simulink library "ddm"  (R2021b)
settings: Solver=VariableStepAuto  StartTime=0.0  StopTime=10.0  RelTol=1e-3
undefined symbols (not defined in the file or in its folder): ENUM_ADASACCSTA_ERROR, ENUM_ADASACCSTA_OFF, ENUM_ADASACCSTA_STANDBY, ENUM_ADASISASTA_OFF, ENUM_ALLOWMOV_ALLOWREADY, ENUM_APS, ENUM_BRKSTA_ERROR, ENUM_BRKSTA_OFF, ENUM_BRKSTA_ON, ENUM_BRKSW_INVALID, ENUM_BRKSW_OFF, ENUM_BRKSW_ON, ENUM_CHGPREACTERRSTA_OBCPRE, ENUM_DCDCFAULTSTA_ANYFAULTLV1, ENUM_DCDCFAULTSTA_ANYFAULTLV2, ENUM_DRIVETRAIN_AWD, ENUM_DRIVETRAIN_FWD, ENUM_DRIVETRAIN_RWD, ENUM_DRSEATSTA_INVALID, ENUM_EDUDRTSTA_NORMAL, ENUM_EPBSTA_APPLIED, ENUM_EPBSTA_RELEASED, ENUM_HVBATTREADYPRE_READY, ENUM_MCUWARN_LV0, ENUM_MCUWARN_LV1, ENUM_MCUWARN_LV2, ENUM_MCUWARN_LV3, ENUM_MCUWARN_NOERROR, ENUM_OBCFAULTSTA_ANYFAULT, ENUM_PAS_R2F2, ENUM_PDFAULT_BATTPDFAIL, ENUM_PDFAULT_DCDCDISABLE, ENUM_PDFAULT_MCUDISABLE, ENUM_PDFAULT_MCUDISCHRG, ENUM_POWERSTA_OFF, ENUM_POWERSTA_ON, ENUM_POWERSTA_READY, ENUM_POWERSTA_STANDBY, ENUM_PRESSINDI_LOW, ENUM_PUFAULT_BATTUPFAIL, ENUM_PUFAULT_DCDCENABLEFAIL, ENUM_PUFAULT_PRECHRGCHKFAIL, ENUM_PUFAULT_SAFETYCHKFAIL, ENUM_PUSTATE_COMPLETED, ENUM_PWRSTASW_OFF, ENUM_PWRSTASW_OFFA, ENUM_PWRSTASW_OFFCHVCHRG, ENUM_PWRSTASW_OFFCLVCHRG, ENUM_PWRSTASW_ON, ENUM_PWRSTASW_ONHVCHRG, ENUM_PWRSTASW_READY, ENUM_PWRSTASW_STANDBY, ENUM_RANGESTA_12IN, ENUM_SHIFTCOMMAND_D, ENUM_SHIFTCOMMAND_N, ENUM_SHIFTCOMMAND_P, ENUM_SHIFTCOMMAND_R, ENUM_VEHMALFUNLV_2ND, ENUM_VEHMALFUNLV_3RD, ENUM_VEHMALFUNLV_4TH ... (+835)
libraries: hcu_lib x750, $bdroot x12, simulink x5
(part 2 of 28)

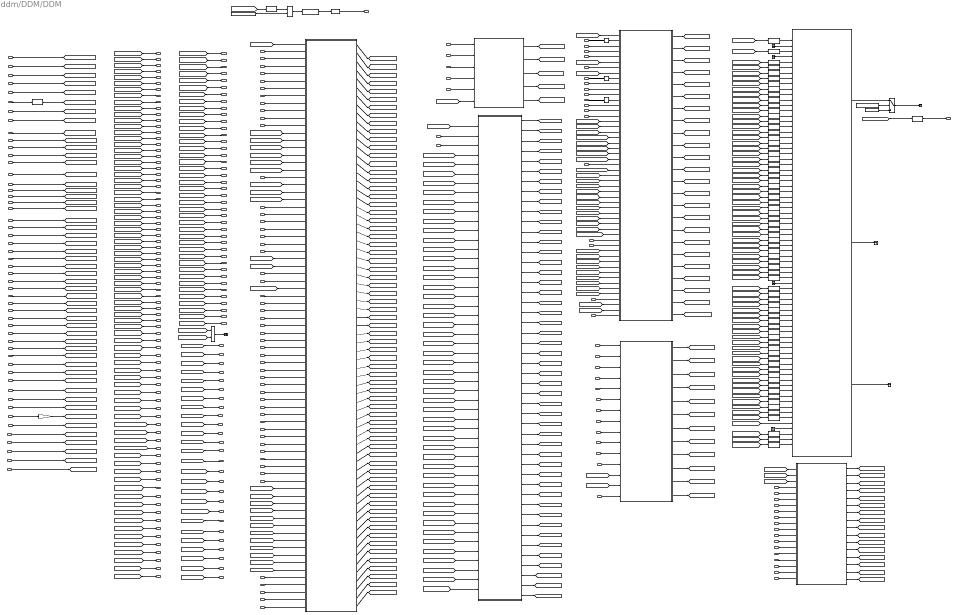
== system ddm/DDM/DDM ==
  task_time_s : Inport
  VINP_CANMsgValidABM1_flg : Inport  Port=2
  VINP_BrkPedalPosSta_enum : Inport  Port=3
  VINP_BrkPedalPos_pct : Inport  Port=4
  VINP_BrkSWSta_flg : Inport  Port=5
  VINP_CANMsgValidESC7_flg : Inport  Port=6
  VINP_CANMsgValidESC1_flg : Inport  Port=7
  VINP_CANMsgValidESC5_flg : Inport  Port=8
  VINP_CANMsgValidFCM2_flg : Inport  Port=9
  VINP_CANMsgValidFCM3_flg : Inport  Port=10
  VINP_CANMsgValidFCM4_flg : Inport  Port=11
  VINP_ADASACCSta_enum : Inport  Port=12
  VINP_VehSpeed_kph : Inport  Port=13
  VINP_ACCRequireAccel_mps2 : Inport  Port=14
  VDDM_ESC7RCErr_flg : Inport  Port=15
  VDDM_ESC7CSErr_flg : Inport  Port=16
  VDDM_ESC1RCErr_flg : Inport  Port=17
  VDDM_ESC1CSErr_flg : Inport  Port=18
  VDDM_ESC5RCErr_flg : Inport  Port=19
  VDDM_ESC5CSErr_flg : Inport  Port=20
  VDDM_FCM2RCErr_flg : Inport  Port=21
  VDDM_FCM2CSErr_flg : Inport  Port=22
  VDDM_FCM3RCErr_flg : Inport  Port=23
  VDDM_FCM3CSErr_flg : Inport  Port=24
  VDDM_FCM4CSErr_flg : Inport  Port=25
  VDDM_C1ABM1RCChk_flg : Inport  Port=26
  VDDM_C1ABM1CSChk_flg : Inport  Port=27
  VINP_CANMsgValidEPAS2_flg : Inport  Port=28
  VINP_EPBSta_enum : Inport  Port=29
  VDDM_FCM5CSErr_flg : Inport  Port=30
  VDDM_FCM5NoCom_flg : Inport  Port=31
  VINP_ADASISASta_enum : Inport  Port=32
  VINP_CANMsgValidBMS1_flg : Inport  Port=33
  VINP_CANMsgValidBMS6_flg : Inport  Port=34
  VINP_CANMsgValidCCU1_flg : Inport  Port=35
  VINP_CANMsgValidCCU2_flg : Inport  Port=36
  VINP_BMSWarn1_flg : Inport  Port=37
  VINP_BMSWarn2_flg : Inport  Port=38
  VINP_BMSWarn3_flg : Inport  Port=39
  VINP_BMSWarn4_flg : Inport  Port=40
  VINP_BMSWarn5_flg : Inport  Port=41
  VINP_BMSWarn6_flg : Inport  Port=42
  VINP_BMSWarn7_flg : Inport  Port=43
  VINP_BMSWarn8_flg : Inport  Port=44
  VINP_DCDCFaultSta_enum : Inport  Port=45
  VINP_OBCFaultSta_enum : Inport  Port=46
  VINP_MCUWarnF_enum : Inport  Port=47
  VINP_MCUWarnR_enum : Inport  Port=48
  VINP_LVBattDet12V_V : Inport  Port=49
  VINP_BMSREADY_flg : Inport  Port=50
  VINP_HVBattReady4Pre_enum : Inport  Port=51
  VINP_HVBContactorSta_flg : Inport  Port=52
  VINP_DCDCReady4Pre_flg : Inport  Port=53
  VINP_DCDCEnabled_flg : Inport  Port=54
  VINP_CANMsgValidBMS2_flg : Inport  Port=55
  VINP_CANMsgValidMCUF1_flg : Inport  Port=56
  VINP_CANMsgValidMCUR1_flg : Inport  Port=57
  VINP_CANMsgValidShifter1_flg : Inport  Port=58
  VINP_FrEDUDrtSta_flg : Inport  Port=59
  VINP_FrEDURealTMTq_Nm : Inport  Port=60
  VINP_RrEDUDrtSta_flg : Inport  Port=61
  VINP_RrEDURealTMTq_Nm : Inport  Port=62
  VDDM_C3BMS6RCChk_flg : Inport  Port=63
  VDDM_C3BMS6CSChk_flg : Inport  Port=64
  VDDM_C3BMS1RCChk_flg : Inport  Port=65
  VDDM_C3BMS1CSChk_flg : Inport  Port=66
  VDDM_C3CCU1RCChk_flg : Inport  Port=67
  VDDM_C3CCU1CSChk_flg : Inport  Port=68
  VDDM_C3CCU2RCChk_flg : Inport  Port=69
  VDDM_C3CCU2CSChk_flg : Inport  Port=70
  VDDM_MCUF1RCErr_flg : Inport  Port=71
  VDDM_MCUF1CSErr_flg : Inport  Port=72
  VDDM_MCUR1RCErr_flg : Inport  Port=73
  VDDM_MCUR1CSErr_flg : Inport  Port=74
  VDDM_Shifter1RCErr_flg : Inport  Port=75
  VDDM_Shifter1CSErr_flg : Inport  Port=76
  VINP_HVBattSOC_pct : Inport  Port=77
  VINP_ShifterHandleCmd_enum : Inport  Port=78
  VPMM_PowerSta_enum : Inport  Port=79
  VPMM_PwrStaSW_enum : Inport  Port=80
  VPMM_PowerUpFault_enum : Inport  Port=81
  VPMM_PowerDownFault_enum : Inport  Port=82
  VPMM_DrivetrainSelect_enum : Inport  Port=83
  VPMM_SafetyChkHLv_flg : Inport  Port=84
  VPMM_SafetyChkMLv_flg : Inport  Port=85
  VPMM_HVChrgPreActionErrSta_enum : Inport  Port=86
  VPMM_MCUReady_flg : Inport  Port=87
  VPMM_MCUReady4Pre_flg : Inport  Port=88
  VPMM_PowerUpState_enum : Inport  Port=89
  VPMM_MCUDCBusMaxVolt_V : Inport  Port=90
  VINP_BrakeSWGPIO_flg : Inport  Port=91
  VINP_BrakeLampSW_flg : Inport  Port=92
  VINP_DrStSW : Inport  Port=93
  VINP_FLAJARSW : Inport  Port=94
  VINP_FRAJARSW : Inport  Port=95
  VINP_RLAJARSW : Inport  Port=96
  VINP_RRAJARSW : Inport  Port=97
  VINP_HoodSW : Inport  Port=98
  VINP_TailgaSW : Inport  Port=99
  VINP_AccelPedal1Vol_V : Inport  Port=100
  VINP_AccelPedal2Vol_V : Inport  Port=101
  VDKC_DKCAuthSta_enum : Inport  Port=102
  VINP_AllowMovThd_OTA_enum : Inport  Port=103
  VINP_Pedal1Ref5V_V : Inport  Port=104
  VINP_Pedal2Ref5V_V : Inport  Port=105
  VINP_AuxBattVolmV_mV : Inport  Port=106
  No_CAN1_BUS_OFF : Inport  Port=107
  No_CAN3_BUS_OFF : Inport  Port=108
  No_CAN4_BUS_OFF : Inport  Port=109
  No_CAN_BUS_OFF : Inport  Port=110
  DTC_clear_request : Inport  Port=111
  VDHP_EAPCRBAD_flg : Inport  Port=112
  VDHP_EAPS12RangeSta_enum : Inport  Port=113
  VBCM_DiagHCrash_flg : Inport  Port=114
  VBCM_DiagFLTS_flg : Inport  Port=115
  VBCM_DiagFRTS_flg : Inport  Port=116
  VBCM_DiagRLTS_flg : Inport  Port=117
  VBCM_DiagRRTS_flg : Inport  Port=118
  VAPM_USSStaFCL_flg : Inport  Port=119
  VAPM_USSStaFML_flg : Inport  Port=120
  VAPM_USSStaFMR_flg : Inport  Port=121
  VAPM_USSStaFCR_flg : Inport  Port=122
  VAPM_USSStaRCL_flg : Inport  Port=123
  VAPM_USSStaRML_flg : Inport  Port=124
  VAPM_USSStaRMR_flg : Inport  Port=125
  VAPM_USSStaRCR_flg : Inport  Port=126
  VAPM_USSStaFLL_flg : Inport  Port=127
  VAPM_USSStaFLR_flg : Inport  Port=128
  VAPM_USSStaRLL_flg : Inport  Port=129
  VAPM_USSStaRLR_flg : Inport  Port=130
  VAPM_SNSRLayout_enum : Inport  Port=131
  VINP_ZoneSpdCtrlMode_enum : Inport  Port=132
  VDDM_ZoneSCPNoCom_flg : Inport  Port=133
  VINP_DrStdAErrSta_enum : Inport  Port=134
  VINP_ZoneDrMalfunLevel_enum : Inport  Port=135
  VINP_CANMsgValidDKC1_flg : Inport  Port=136
  VINP_CANMsgValidDKC2_flg : Inport  Port=137
  VVMC_ADASActive_flg : Inport  Port=138
  VTQR_FrTMTqReq_Nm : Inport  Port=139
  VTQR_RrTMTqReq_Nm : Inport  Port=140
  VTPM_LFBatwarn_flg : Inport  Port=141
  VTPM_RFBatwarn_flg : Inport  Port=142
  VTPM_LRBatwarn_flg : Inport  Port=143
  VTPM_RRBatwarn_flg : Inport  Port=144
  VTPM_LFPressIndi_enum : Inport  Port=145
  VTPM_RFPressIndi_enum : Inport  Port=146
  VTPM_LRPressIndi_enum : Inport  Port=147
  VTPM_RRPressIndi_enum : Inport  Port=148
  VTPM_LFWheelTmpIndi_flg : Inport  Port=149
  VTPM_RFWheelTmpIndi_flg : Inport  Port=150
  VTPM_LRWheelTmpIndi_flg : Inport  Port=151
  VTPM_RRWheelTmpIndi_flg : Inport  Port=152
  VTPM_LFSensorFail_flg : Inport  Port=153
  VTPM_RFSensorFail_flg : Inport  Port=154
  VTPM_LRSensorFail_flg : Inport  Port=155
  VTPM_RRSensorFail_flg : Inport  Port=156
  VTQD_ActParkRequest_flg : Inport  Port=157
  APM : Subsystem
  BCM : Subsystem
  Chart : Stateflow chart  TreatAsAtomicUnit=on
      settings: PortSchema="{\"entries\":[{\"content\":{\"sides\":[{\"content\":{\"connectorIds\":[]},\"type\":\"ConnectorPlacement.EquallySpacedRectSide\",\"uuid\":\"5c49d68c-3a13-4722-ae51-60c531d65ae1\"},{\"content\":{\"connectorIds\":[],\"side\":\"RIGHT\"},\"type\":\"ConnectorPlacement.EquallySpacedRectSide\",\"uuid\":\"1499f12d-58db-4e43-953b-81e532540c9e\"},{\"content\":{\"connectorIds\":[\"Out1\",\"Out2\",\"Out3\"],\"side\":\"TOP\"},\"type\":\"ConnectorPlacement.EquallySpacedRectSide\",\"uuid\":\"b40fb5a5-59a6-496c-b268-75370edec7d4\"},{\"content\":{\"connectorIds\":[\"In2\",\"In3\",\"In4\",\"In5\",\"In6\",\"In7\",\"In8\",\"In9\",\"In10\",\"In11\",\"In12\",\"In13\",\"In14\",\"In15\",\"In16\",\"In17\",\"In18\",\"In19\",\"In20\",\"In21\",\"In22\",\"In23\",\"In24\",\"In25\",\"In26\",\"In27\",\"In28\",\"In29\",\"In30\",\"In31\",\"In32\",\"In33\",\"In34\",\"In35\",\"In36\",\"In37\",\"In38\",\"In39\",\"In40\",\"In41\",\"In42\",\"In43\",\"In44\",\"In45\",\"In46\",\"In47\",\"In48\",\"In49\",\"In50\",\"In51\",\"In52\",\"In1\",\"In53\",\"In54\",\"In55\",\"In56\",\"In57\",\"In58\",\"In59\",\"In60\",\"In61\",\"In62\",\"In63\",\"In64\",\"In65\",\"In66\",\"In67\",\"In68\",\"In69\",\"In70\",\"In71\",\"In72\",\"In73\",\"In74\",\"In75\",\"In76\"],\"side\":\"BOTTOM\"},\"type\":\"ConnectorPlacement.EquallySpacedRectSide\",\"uuid\":\"7a3e18bf-6f06-4df1-889c-341cd16aa4bd\"}]},\"type\":\"ConnectorPlacement.EquallySpacedConnector\",\"uuid\":\"c096d691-37a2-471f-9d84-793135a13589\"}],\"packageUris\":[\"http://schema.mathworks.com/mf0/Connector/R2020b\"],\"version\":\"1.0\"}"
  Constant : Constant  Value=ENUM_PWRSTASW_READY
  Constant1 : Constant  Value=ZERO_INT
  Constant15 : Constant  Value=KDDM_VehMalfunLevelSW_flg
  Data Type Conversion{,1..48,50..72} (72 alike) : DataTypeConversion  OutDataTypeStr=boolean
  Data Type Conversion49 : DataTypeConversion  OutDataTypeStr=uint8
  Data Type Conversion73 : DataTypeConversion  OutDataTypeStr=uint8
  Detect Increase : simulink/Logic and Bit Operations/Detect Increase  vinit=0.0  OutDataTypeStr=boolean
  Equal : RelationalOperator  Operator===  OutDataTypeStr=boolean  RndMeth=Simplest
  Gain : Gain  Gain=XX2KXX
  Ground{1,3..4,26} (4 alike) : Ground
  Latch : hcu_lib/Basic_Blocks/Latch
  Logical Operator : Logic  Operator=NOT  AllPortsSameDT=off  OutDataTypeStr=boolean
  Logical Operator1 : Logic  Operator=NOT  AllPortsSameDT=off  OutDataTypeStr=boolean
  Logical Operator2 : Logic  Operator=NOT  AllPortsSameDT=off  OutDataTypeStr=boolean
  Logical Operator5 : Logic  Operator=OR  AllPortsSameDT=off  OutDataTypeStr=boolean
  PMM : Subsystem
  Switch : Switch  Criteria=u2 > Threshold
  TPM : Subsystem
  TQD : Subsystem
  Terminator{,1..3} (4 alike) : Terminator
  VMC_DDM : Subsystem
  VDDM_C3BMS6RCDTC_raw32 : Outport
  VDDM_C3BMS6CSDTC_raw32 : Outport  Port=2
  VDDM_C3BMS6LCDTC_raw32 : Outport  Port=3
  VDDM_C3BMS1RCDTC_raw32 : Outport  Port=4
  VDDM_C3BMS1CSDTC_raw32 : Outport  Port=5
  VDDM_C3BMS1LCDTC_raw32 : Outport  Port=6
  VDDM_C3CCU1RCDTC_raw32 : Outport  Port=7
  VDDM_C3CCU1CSDTC_raw32 : Outport  Port=8
  VDDM_C3CCU1LCDTC_raw32 : Outport  Port=9
  VDDM_C3CCU2RCDTC_raw32 : Outport  Port=10
  VDDM_C3CCU2CSDTC_raw32 : Outport  Port=11
  VDDM_C3CCU2LCDTC_raw32 : Outport  Port=12
  VDDM_C1ABM1RCDTC_raw32 : Outport  Port=13
  VDDM_C1ABM1CSDTC_raw32 : Outport  Port=14
  VDDM_C1ABM1LCDTC_raw32 : Outport  Port=15
  VDDM_Lv1ErrDTC_raw32 : Outport  Port=16
  VDDM_Lv2ErrDTC_raw32 : Outport  Port=17
  VDDM_Lv3ErrDTC_raw32 : Outport  Port=18
  VDDM_Lv4ErrDTC_raw32 : Outport  Port=19
  VDDM_BrkSWErrDTC_raw32 : Outport  Port=20
  VDDM_BrkSWNoBacDTC_raw32 : Outport  Port=21
  VDDM_KeyAuthDTC_raw32 : Outport  Port=22
  VDDM_ONtoRdyDTC_raw32 : Outport  Port=23
  VDDM_HVB4PreDTC_raw32 : Outport  Port=24
  VDDM_MCU4PreDTC_raw32 : Outport  Port=25
  VDDM_DCDC4PreDTC_raw32 : Outport  Port=26
  VDDM_HVRlyCloDTC_raw32 : Outport  Port=27
  VDDM_BMSRdyDTC_raw32 : Outport  Port=28
  VDDM_DCDCEnaDTC_raw32 : Outport  Port=29
  VDDM_HiLvSaChkDTC_raw32 : Outport  Port=30
  VDDM_MidLvSaChkDTC_raw32 : Outport  Port=31
  VDDM_MCUDisDTC_raw32 : Outport  Port=32
  VDDM_DCDCDisDTC_raw32 : Outport  Port=33
  VDDM_HVRlyOpDTC_raw32 : Outport  Port=34
  VDDM_MCUActDTC_raw32 : Outport  Port=35
  VDDM_OBC4PreDTC_raw32 : Outport  Port=36
  VDDM_IniLVLoDTC_raw32 : Outport  Port=37
  VDDM_LVSupLoDTC_raw32 : Outport  Port=38
  VDDM_LVSupHiDTC_raw32 : Outport  Port=39
  VDDM_DrStSWDTC_raw32 : Outport  Port=40
  VDDM_FLDoorSWDTC_raw32 : Outport  Port=41
  VDDM_RLDoorSWDTC_raw32 : Outport  Port=42
  VDDM_FRDoorSWDTC_raw32 : Outport  Port=43
  VDDM_RRDoorSWDTC_raw32 : Outport  Port=44
  VDDM_HoodSWDTC_raw32 : Outport  Port=45
  VDDM_TailgaSWDTC_raw32 : Outport  Port=46
  VDDM_VehMalfunLevel_enum : Outport  Port=47
  VDDM_APS1SigOoRDTC_raw32 : Outport  Port=48
  VDDM_APS2SigOoRDTC_raw32 : Outport  Port=49
  VDDM_APSCorrErrDTC_raw32 : Outport  Port=50
  VDDM_MCUF1NoComDTC_raw32 : Outport  Port=51
  VDDM_MCUR1NoComDTC_raw32 : Outport  Port=52
  VDDM_Shifter1NoComDTC_raw32 : Outport  Port=53
  VDDM_ESC7NoComDTC_raw32 : Outport  Port=54
  VDDM_ESC1NoComDTC_raw32 : Outport  Port=55
  VDDM_ESC5NoComDTC_raw32 : Outport  Port=56
  VDDM_EnterNewOperCyc_flg : Outport  Port=57
  VDDM_DiagHCrashDTC_raw32 : Outport  Port=58
  VDDM_DiagFLTSDTC_raw32 : Outport  Port=59
  VDDM_DiagFRTSDTC_raw32 : Outport  Port=60
  VDDM_DiagRLTSDTC_raw32 : Outport  Port=61
  VDDM_DiagRRTSDTC_raw32 : Outport  Port=62
  VDDM_FCLUSSDTC_raw32 : Outport  Port=63
  VDDM_FMLUSSDTC_raw32 : Outport  Port=64
  VDDM_FMRUSSDTC_raw32 : Outport  Port=65
  VDDM_FCRUSSDTC_raw32 : Outport  Port=66
  VDDM_RCLUSSDTC_raw32 : Outport  Port=67
  VDDM_RMLUSSDTC_raw32 : Outport  Port=68
  VDDM_RMRUSSDTC_raw32 : Outport  Port=69
  VDDM_RCRUSSDTC_raw32 : Outport  Port=70
  VDDM_FLLUSSDTC_raw32 : Outport  Port=71
  VDDM_FLRUSSDTC_raw32 : Outport  Port=72
  VDDM_RLLUSSDTC_raw32 : Outport  Port=73
  VDDM_RLRUSSDTC_raw32 : Outport  Port=74
  VDDM_FCM2NoComDTC_raw32 : Outport  Port=75
  VDDM_FCM2RCErrDTC_raw32 : Outport  Port=76
  VDDM_FCM2CSErrDTC_raw32 : Outport  Port=77
  VDDM_FCM3NoComDTC_raw32 : Outport  Port=78
  VDDM_FCM3RCErrDTC_raw32 : Outport  Port=79
  VDDM_FCM3CSErrDTC_raw32 : Outport  Port=80
  VDDM_FCM4NoComDTC_raw32 : Outport  Port=81
  VDDM_FCM4CSErrDTC_raw32 : Outport  Port=82
  VDDM_FCM5NoComDTC_raw32 : Outport  Port=83
  VDDM_FCM5CSErrDTC_raw32 : Outport  Port=84
  VDDM_ZoneSCPNoComDTC_raw32 : Outport  Port=85
  VDDM_BMSSigErrDetDTC_raw32 : Outport  Port=86
  VDDM_FCMACCSigErrDetDTC_raw32 : Outport  Port=87
  VDDM_FrMCUSigErrDetDTC_raw32 : Outport  Port=88
  VDDM_RrMCUSigErrDetDTC_raw32 : Outport  Port=89
  VDDM_CCUSigErrDetDTC_raw32 : Outport  Port=90
  VDDM_ACCAccelCmdErrDetDTC_raw32 : Outport  Port=91
  VDDM_ACCMalfuncDetDTC_raw32 : Outport  Port=92
  VDDM_CCMalfuncDetDTC_raw32 : Outport  Port=93
  VDDM_MSAMalfuncDetDTC_raw32 : Outport  Port=94
  VDDM_ISAMalfuncDetDTC_raw32 : Outport  Port=95
  VDDM_MCUF1RCErrDTC_raw32 : Outport  Port=96
  VDDM_MCUR1RCErrDTC_raw32 : Outport  Port=97
  VDDM_MCUF1CSErrDTC_raw32 : Outport  Port=98
  VDDM_MCUR1CSErrDTC_raw32 : Outport  Port=99
  VDDM_Shifter1RCErrDTC_raw32 : Outport  Port=100
  VDDM_Shifter1CSErrDTC_raw32 : Outport  Port=101
  VDDM_ESC7RCErrDTC_raw32 : Outport  Port=102
  VDDM_ESC7CSErrDTC_raw32 : Outport  Port=103
  VDDM_ESC1RCErrDTC_raw32 : Outport  Port=104
  VDDM_ESC1CSErrDTC_raw32 : Outport  Port=105
  VDDM_ESC5RCErrDTC_raw32 : Outport  Port=106
  VDDM_ESC5CSErrDTC_raw32 : Outport  Port=107
  VDDM_FrMCUTqErrDTC_raw32 : Outport  Port=108
  VDDM_RrMCUTqErrDTC_raw32 : Outport  Port=109
  VDDM_LFBatwarnDTC_raw32 : Outport  Port=110
  VDDM_RFBatwarnDTC_raw32 : Outport  Port=111
  VDDM_LRBatwarnDTC_raw32 : Outport  Port=112
  VDDM_RRBatwarnDTC_raw32 : Outport  Port=113
  VDDM_LFPressIndiDTC_raw32 : Outport  Port=114
  VDDM_RFPressIndiDTC_raw32 : Outport  Port=115
  VDDM_LRPressIndiDTC_raw32 : Outport  Port=116
  VDDM_RRPressIndiDTC_raw32 : Outport  Port=117
  VDDM_LFWheelTmpHighDTC_raw32 : Outport  Port=118
  VDDM_RFWheelTmpHighDTC_raw32 : Outport  Port=119
  VDDM_LRWheelTmpHighDTC_raw32 : Outport  Port=120
  VDDM_RRWheelTmpHighDTC_raw32 : Outport  Port=121
  VDDM_LFSensorFailDTC_raw32 : Outport  Port=122
  VDDM_RFSensorFailDTC_raw32 : Outport  Port=123
  VDDM_LRSensorFailDTC_raw32 : Outport  Port=124
  VDDM_RRSensorFailDTC_raw32 : Outport  Port=125
  VDDM_C1EPAS2LCDTC_raw32 : Outport  Port=126
  VDDM_5vAPS1PwrErrDTC_raw32 : Outport  Port=127
  VDDM_5vAPS2PwrErrDTC_raw32 : Outport  Port=128
  VDDM_EPBLockTODTC_raw32 : Outport  Port=129
  VDDM_EPBUnlockTODTC_raw32 : Outport  Port=130
  VDDM_HVRlyOpCFS_flg : Outport  Port=131
  VDDM_MCUActCFS_flg : Outport  Port=132
  VDDM_VCUACCErr_flg : Outport  Port=133
  VDDM_VCUISAErr_flg : Outport  Port=134
  VDDM_HVRlyOpFail_flg : Outport  Port=135
  VDDM_MCUActDisFail_flg : Outport  Port=136
  VDDM_VCUBrkSWSta_enum : Outport  Port=137
  VDDM_DrSeatSta_enum : Outport  Port=138
  VDDM_VCUFLDoorSta_flg : Outport  Port=139
  VDDM_VCUFRDoorSta_flg : Outport  Port=140
  VDDM_VCURLDoorSta_flg : Outport  Port=141
  VDDM_VCURRDoorSta_flg : Outport  Port=142
  VDDM_SysAllowReadySta_flg : Outport  Port=143
  VDDM_VCUHoodSWSta_flg : Outport  Port=144
  VDDM_VCUTailgateSWSta_flg : Outport  Port=145
  VDDM_LimpHomeActTmp_flg : Outport  Port=146
  VDDM_EDriveSysErr_VCUErrTmp_flg : Outport  Port=147
  wires:
  [VDDM_VCUTailgateSWSta_flg] -> VDDM_VCUTailgateSWSta_flg/1
  [VDDM_VCUHoodSWSta_flg] -> VDDM_VCUHoodSWSta_flg/1
  [VDDM_VCURRDoorSta_flg] -> VDDM_VCURRDoorSta_flg/1
  [VDDM_VCURLDoorSta_flg] -> VDDM_VCURLDoorSta_flg/1
  [VDDM_VCUFRDoorSta_flg] -> VDDM_VCUFRDoorSta_flg/1
  [VDDM_VCUFLDoorSta_flg] -> VDDM_VCUFLDoorSta_flg/1
  [VDDM_DrSeatSta_enum] -> VDDM_DrSeatSta_enum/1
  [VDDM_VCUBrkSWSta_enum] -> VDDM_VCUBrkSWSta_enum/1
  [VDDM_MCUActDisFail_flg] -> VDDM_MCUActDisFail_flg/1
  [VDDM_HVRlyOpFail_flg] -> VDDM_HVRlyOpFail_flg/1
  VPMM_MCUDCBusMaxVolt_V/1 -> PMM/75(VPMM_MCUDCBusMaxVolt_V)
  [VDDM_HVRlyOpCFS_flg] -> VDDM_HVRlyOpCFS_flg/1
  [VDDM_MCUActCFS_flg] -> VDDM_MCUActCFS_flg/1
  PMM/67(VDDM_MCUActCFS_flg) -> [VDDM_MCUActCFS_flg]
  PMM/66(VDDM_HVRlyOpCFS_flg) -> [VDDM_HVRlyOpCFS_flg]
  VINP_ZoneDrMalfunLevel_enum/1 -> [VINP_ZoneDrMalfunLevel_enum]
  PMM/65(VDDM_MCUActDisFail_flg) -> [VDDM_MCUActDisFail_flg]
  PMM/64(VDDM_HVRlyOpFail_flg) -> [VDDM_HVRlyOpFail_flg]
  PMM/63(VDDM_VCUTailgateSWSta_flg) -> [VDDM_VCUTailgateSWSta_flg]
  PMM/62(VDDM_VCUHoodSWSta_flg) -> [VDDM_VCUHoodSWSta_flg]
  PMM/61(VDDM_VCURRDoorSta_flg) -> [VDDM_VCURRDoorSta_flg]
  PMM/60(VDDM_VCURLDoorSta_flg) -> [VDDM_VCURLDoorSta_flg]
  PMM/59(VDDM_VCUFRDoorSta_flg) -> [VDDM_VCUFRDoorSta_flg]
  PMM/58(VDDM_VCUFLDoorSta_flg) -> [VDDM_VCUFLDoorSta_flg]
  PMM/57(VDDM_DrSeatSta_enum) -> [VDDM_DrSeatSta_enum]
  PMM/56(VDDM_SysAllowReadySta_flg) -> [VDDM_SysAllowReadySta_flg]
  PMM/55(VDDM_VCUBrkSWSta_enum) -> [VDDM_VCUBrkSWSta_enum]
  [VDDM_EPBUnlockTODTC_raw32] -> VDDM_EPBUnlockTODTC_raw32/1
  [VDDM_EPBLockTODTC_raw32] -> VDDM_EPBLockTODTC_raw32/1
  [VDDM_EPBUnlockTODTC_raw32] -> Data Type Conversion72/1
  [VDDM_EPBLockTODTC_raw32] -> Data Type Conversion71/1
  Data Type Conversion72/1 -> Chart/29(VDDM_EPBUnlockTOCFS_flg)
  Data Type Conversion71/1 -> Chart/28(VDDM_EPBLockTOCFS_flg)
  VINP_ShifterHandleCmd_enum/1 -> [VINP_ShifterHandleCmd_enum]
  VINP_EPBSta_enum/1 -> [VINP_EPBSta_enum]
  VTQD_ActParkRequest_flg/1 -> [VTQD_ActParkRequest_flg]
  TQD/42(VDDM_EPBUnlockTODTC_raw32) -> [VDDM_EPBUnlockTODTC_raw32]
  TQD/41(VDDM_EPBLockTODTC_raw32) -> [VDDM_EPBLockTODTC_raw32]
  [VINP_ShifterHandleCmd_enum] -> TQD/43(VINP_ShifterHandleCmd_enum)
  [VINP_EPBSta_enum] -> TQD/42(VINP_EPBSta_enum)
  [VTQD_ActParkRequest_flg] -> TQD/41(VTQD_ActParkRequest_flg)
  [VINP_LVBattDet12V_V] -> TQD/40(VDDM_AuxBattVolV_V)
  Gain/1 -> [VDDM_AuxBattVolV_V]
  VINP_AuxBattVolmV_mV/1 -> Gain/1
  [VDDM_5vAPS2PwrErrDTC_raw32] -> VDDM_5vAPS2PwrErrDTC_raw32/1
  [VDDM_5vAPS1PwrErrDTC_raw32] -> VDDM_5vAPS1PwrErrDTC_raw32/1
  Data Type Conversion69/1 -> Chart/4(VDDM_5vAPS2OoCFS_flg)
  [VDDM_5vAPS2PwrErrDTC_raw32] -> Data Type Conversion69/1
  Data Type Conversion70/1 -> Chart/2(VDDM_5vAPS1OoCFS_flg)
  [VDDM_5vAPS1PwrErrDTC_raw32] -> Data Type Conversion70/1
  TQD/40(VDDM_5vAPS2PwrErrDTC_raw32) -> [VDDM_5vAPS2PwrErrDTC_raw32]
  TQD/39(VDDM_5vAPS1PwrErrDTC_raw32) -> [VDDM_5vAPS1PwrErrDTC_raw32]
  [VINP_HVBattSOC_pct] -> TQD/39(VINP_HVBattSOC_pct)
  VINP_HVBattSOC_pct/1 -> [VINP_HVBattSOC_pct]
  [VINP_Pedal2Ref5V_V] -> TQD/38(VINP_Pedal2Ref5V_V)
  [VINP_Pedal1Ref5V_V] -> TQD/37(VINP_Pedal1Ref5V_V)
  VINP_Pedal2Ref5V_V/1 -> [VINP_Pedal2Ref5V_V]
  VINP_Pedal1Ref5V_V/1 -> [VINP_Pedal1Ref5V_V]
  [VDDM_RRSensorFailDTC_raw32] -> VDDM_RRSensorFailDTC_raw32/1
  [VDDM_LRSensorFailDTC_raw32] -> VDDM_LRSensorFailDTC_raw32/1
  [VDDM_RFSensorFailDTC_raw32] -> VDDM_RFSensorFailDTC_raw32/1
  [VDDM_LFSensorFailDTC_raw32] -> VDDM_LFSensorFailDTC_raw32/1
  TPM/15(VDDM_LRSensorFailDTC_raw32) -> [VDDM_LRSensorFailDTC_raw32]
  TPM/14(VDDM_RFSensorFailDTC_raw32) -> [VDDM_RFSensorFailDTC_raw32]
  TPM/16(VDDM_RRSensorFailDTC_raw32) -> [VDDM_RRSensorFailDTC_raw32]
  TPM/13(VDDM_LFSensorFailDTC_raw32) -> [VDDM_LFSensorFailDTC_raw32]
  VTPM_LFSensorFail_flg/1 -> TPM/16(VTPM_LFSensorFail_flg)
  VTPM_RFSensorFail_flg/1 -> TPM/17(VTPM_RFSensorFail_flg)
  VTPM_LRSensorFail_flg/1 -> TPM/18(VTPM_LRSensorFail_flg)
  VTPM_RRSensorFail_flg/1 -> TPM/19(VTPM_RRSensorFail_flg)
  VAPM_SNSRLayout_enum/1 -> APM/15(VAPM_SNSRLayout_enum)
  [VDDM_C1EPAS2LCDTC_raw32] -> VDDM_C1EPAS2LCDTC_raw32/1
  PMM/54(VDDM_C1EPAS2LCDTC_raw32) -> [VDDM_C1EPAS2LCDTC_raw32]
  [VDDM_RRWheelTmpHighDTC_raw32] -> VDDM_RRWheelTmpHighDTC_raw32/1
  [VDDM_LRWheelTmpHighDTC_raw32] -> VDDM_LRWheelTmpHighDTC_raw32/1
  [VDDM_RFWheelTmpHighDTC_raw32] -> VDDM_RFWheelTmpHighDTC_raw32/1
  [VDDM_LFWheelTmpHighDTC_raw32] -> VDDM_LFWheelTmpHighDTC_raw32/1
  [VDDM_RRPressIndiDTC_raw32] -> VDDM_RRPressIndiDTC_raw32/1
  [VDDM_LRPressIndiDTC_raw32] -> VDDM_LRPressIndiDTC_raw32/1
  [VDDM_RFPressIndiDTC_raw32] -> VDDM_RFPressIndiDTC_raw32/1
  [VDDM_LFPressIndiDTC_raw32] -> VDDM_LFPressIndiDTC_raw32/1
  TPM/12(VDDM_RRWheelTmpHighDTC_raw32) -> [VDDM_RRWheelTmpHighDTC_raw32]
  TPM/11(VDDM_LRWheelTmpHighDTC_raw32) -> [VDDM_LRWheelTmpHighDTC_raw32]
  TPM/10(VDDM_RFWheelTmpHighDTC_raw32) -> [VDDM_RFWheelTmpHighDTC_raw32]
  TPM/9(VDDM_LFWheelTmpHighDTC_raw32) -> [VDDM_LFWheelTmpHighDTC_raw32]
  TPM/8(VDDM_RRPressIndiDTC_raw32) -> [VDDM_RRPressIndiDTC_raw32]
  TPM/7(VDDM_LRPressIndiDTC_raw32) -> [VDDM_LRPressIndiDTC_raw32]
  TPM/6(VDDM_RFPressIndiDTC_raw32) -> [VDDM_RFPressIndiDTC_raw32]
  TPM/5(VDDM_LFPressIndiDTC_raw32) -> [VDDM_LFPressIndiDTC_raw32]
  VTPM_RRPressIndi_enum/1 -> TPM/11(VTPM_RRPressIndi_enum)
  VTPM_LRPressIndi_enum/1 -> TPM/10(VTPM_LRPressIndi_enum)
  VTPM_RFWheelTmpIndi_flg/1 -> TPM/13(VTPM_RFWheelTmpIndi_flg)
  VTPM_LFPressIndi_enum/1 -> TPM/8(VTPM_LFPressIndi_enum)
  VTPM_LFWheelTmpIndi_flg/1 -> TPM/12(VTPM_LFWheelTmpIndi_flg)
  VTPM_RFPressIndi_enum/1 -> TPM/9(VTPM_RFPressIndi_enum)
  VTPM_RRWheelTmpIndi_flg/1 -> TPM/15(VTPM_RRWheelTmpIndi_flg)
  VTPM_LRWheelTmpIndi_flg/1 -> TPM/14(VTPM_LRWheelTmpIndi_flg)
  VINP_CANMsgValidEPAS2_flg/1 -> PMM/74(VINP_CANMsgValidEPAS2_flg)
  [VINP_MCUWarnR_enum] -> TQD/36(VINP_MCUWarnR_enum)
  [VINP_MCUWarnF_enum] -> TQD/35(VINP_MCUWarnF_enum)
  Logical Operator2/1 -> VMC_DDM/13(VDDM_FCM4NoCom_flg)
  Logical Operator1/1 -> VMC_DDM/9(VDDM_FCM3NoCom_flg)
  Logical Operator/1 -> VMC_DDM/2(VDDM_FCM2NoCom_flg)
  [VDDM_RRBatwarnDTC_raw32] -> VDDM_RRBatwarnDTC_raw32/1
  [VDDM_LRBatwarnDTC_raw32] -> VDDM_LRBatwarnDTC_raw32/1
  [VDDM_RFBatwarnDTC_raw32] -> VDDM_RFBatwarnDTC_raw32/1
  [VDDM_LFBatwarnDTC_raw32] -> VDDM_LFBatwarnDTC_raw32/1
  TPM/4(VDDM_RRBatwarnDTC_raw32) -> [VDDM_RRBatwarnDTC_raw32]
  TPM/3(VDDM_LRBatwarnDTC_raw32) -> [VDDM_LRBatwarnDTC_raw32]
  TPM/2(VDDM_RFBatwarnDTC_raw32) -> [VDDM_RFBatwarnDTC_raw32]
  TPM/1(VDDM_LFBatwarnDTC_raw32) -> [VDDM_LFBatwarnDTC_raw32]
  VTPM_RRBatwarn_flg/1 -> TPM/7(VTPM_RRBatwarn_flg)
  VTPM_LRBatwarn_flg/1 -> TPM/6(VTPM_LRBatwarn_flg)
  VTPM_RFBatwarn_flg/1 -> TPM/5(VTPM_RFBatwarn_flg)
  VTPM_LFBatwarn_flg/1 -> TPM/4(VTPM_LFBatwarn_flg)
  [DTC_clear_request] -> TPM/3(DTC_clear_request)
  [VPMM_PowerSta_enum] -> TPM/2(VPMM_PowerSta_enum)
  [task_time_s] -> TPM/1(task_time_s)
  PMM/53(VDDM_C3CCU2RCCFS_flg) -> [VDDM_C3CCU2RCCFS_flg]
  PMM/52(VDDM_C3CCU2LCCFS_flg) -> [VDDM_C3CCU2LCCFS_flg]
  PMM/51(VDDM_C3CCU2CSCFS_flg) -> [VDDM_C3CCU2CSCFS_flg]
  PMM/50(VDDM_C3BMS6LCCFS_flg) -> [VDDM_C3BMS6LCCFS_flg]
  PMM/49(VDDM_C3BMS6RCCFS_flg) -> [VDDM_C3BMS6RCCFS_flg]
  PMM/48(VDDM_C3BMS6CSCFS_flg) -> [VDDM_C3BMS6CSCFS_flg]
  [VDDM_Shifter1RCErrDTC_raw32] -> Data Type Conversion68/1
  [VDDM_Shifter1CSErrDTC_raw32] -> Data Type Conversion67/1
  [VDDM_ESC1RCErrDTC_raw32] -> Data Type Conversion66/1
  [VDDM_ESC1CSErrDTC_raw32] -> Data Type Conversion65/1
  [VDDM_ESC5RCErrDTC_raw32] -> Data Type Conversion64/1
  [VDDM_ESC5CSErrDTC_raw32] -> Data Type Conversion63/1
  [VDDM_ESC7CSErrDTC_raw32] -> Data Type Conversion62/1
  [VDDM_ESC7RCErrDTC_raw32] -> Data Type Conversion61/1
  [VDDM_MCUR1RCErrCFS_flg] -> Data Type Conversion60/1
  [VDDM_MCUR1CSErrDTC_raw32] -> Data Type Conversion59/1
  [VDDM_MCUF1RCErrDTC_raw32] -> Data Type Conversion58/1
  [VDDM_MCUF1CSErrDTC_raw32] -> Data Type Conversion57/1
  [VDDM_ESC7RCErrDTC_raw32] -> VDDM_ESC7RCErrDTC_raw32/1
  [VDDM_MCUF1CSErrDTC_raw32] -> VDDM_MCUF1CSErrDTC_raw32/1
  [VDDM_Shifter1CSErrDTC_raw32] -> VDDM_Shifter1CSErrDTC_raw32/1
  [VDDM_MCUR1RCErrDTC_raw32] -> VDDM_MCUR1RCErrDTC_raw32/1
  [VDDM_ESC1RCErrDTC_raw32] -> VDDM_ESC1RCErrDTC_raw32/1
  [VDDM_ESC7CSErrDTC_raw32] -> VDDM_ESC7CSErrDTC_raw32/1
  [VDDM_ESC5RCErrDTC_raw32] -> VDDM_ESC5RCErrDTC_raw32/1
  [VDDM_Shifter1RCErrDTC_raw32] -> VDDM_Shifter1RCErrDTC_raw32/1
  [VDDM_MCUR1CSErrDTC_raw32] -> VDDM_MCUR1CSErrDTC_raw32/1
  [VDDM_RrMCUTqErrDTC_raw32] -> VDDM_RrMCUTqErrDTC_raw32/1
  [VDDM_ESC5CSErrDTC_raw32] -> VDDM_ESC5CSErrDTC_raw32/1
  [VDDM_FrMCUTqErrDTC_raw32] -> VDDM_FrMCUTqErrDTC_raw32/1
  [VDDM_ESC1CSErrDTC_raw32] -> VDDM_ESC1CSErrDTC_raw32/1
  [VDDM_MCUF1RCErrDTC_raw32] -> VDDM_MCUF1RCErrDTC_raw32/1
  VDDM_ESC1RCErr_flg/1 -> [VDDM_ESC1RCErr_flg]
  VDDM_ESC7CSErr_flg/1 -> [VDDM_ESC7CSErr_flg]
  VTQR_RrTMTqReq_Nm/1 -> [VTQR_RrTMTqReq_Nm]
  VDDM_ESC5CSErr_flg/1 -> [VDDM_ESC5CSErr_flg]
  VDDM_Shifter1CSErr_flg/1 -> [VDDM_Shifter1CSErr_flg]
  VDDM_MCUF1RCErr_flg/1 -> [VDDM_MCUF1RCErr_flg]
  VINP_FrEDUDrtSta_flg/1 -> [VINP_FrEDUDrtSta_flg]
  VDDM_ESC1CSErr_flg/1 -> [VDDM_ESC1CSErr_flg]
  VDDM_MCUR1CSErr_flg/1 -> [VDDM_MCUR1CSErr_flg]
  VTQR_FrTMTqReq_Nm/1 -> [VTQR_FrTMTqReq_Nm]
  VDDM_MCUF1CSErr_flg/1 -> [VDDM_MCUF1CSErr_flg]
  VINP_RrEDURealTMTq_Nm/1 -> [VINP_RrEDURealTMTq_Nm]
  VDDM_ESC5RCErr_flg/1 -> [VDDM_ESC5RCErr_flg]
  VDDM_Shifter1RCErr_flg/1 -> [VDDM_Shifter1RCErr_flg]
  VDDM_MCUR1RCErr_flg/1 -> [VDDM_MCUR1RCErr_flg]
  VINP_FrEDURealTMTq_Nm/1 -> [VINP_FrEDURealTMTq_Nm]
  VDDM_ESC7RCErr_flg/1 -> [VDDM_ESC7RCErr_flg]
  VINP_RrEDUDrtSta_flg/1 -> [VINP_RrEDUDrtSta_flg]
  [VDDM_ESC5CSErrCFS_flg] -> VMC_DDM/49(VDDM_ESC5CSErrCFS_flg)
  [VDDM_ESC5RCErrCFS_flg] -> VMC_DDM/48(VDDM_ESC5RCErrCFS_flg)
  [VDDM_ESC1CSErrCFS_flg] -> VMC_DDM/46(VDDM_ESC1CSErrCFS_flg)
  [VDDM_ESC1RCErrCFS_flg] -> VMC_DDM/45(VDDM_ESC1RCErrCFS_flg)
  [VDDM_ESC7CSErrCFS_flg] -> VMC_DDM/43(VDDM_ESC7CSErrCFS_flg)
  [VDDM_ESC7RCErrCFS_flg] -> VMC_DDM/42(VDDM_ESC7RCErrCFS_flg)
  [VDDM_MCUR1CSErrCFS_flg] -> VMC_DDM/34(VDDM_MCUR1CSErrCFS_flg)
  [VDDM_MCUR1RCErrCFS_flg] -> VMC_DDM/33(VDDM_MCUR1RCErrCFS_flg)
  [VDDM_MCUF1CSErrCFS_flg] -> VMC_DDM/29(VDDM_MCUF1CSErrCFS_flg)
  [VDDM_MCUF1RCErrCFS_flg] -> VMC_DDM/28(VDDM_MCUF1RCErrCFS_flg)
  TQD/38(VDDM_ESC5CSErrCFS_flg) -> [VDDM_ESC5CSErrCFS_flg]
  TQD/37(VDDM_ESC5RCErrCFS_flg) -> [VDDM_ESC5RCErrCFS_flg]
  TQD/36(VDDM_ESC5NoComCFS_flg) -> [VDDM_ESC5NoComCFS_flg]
  TQD/35(VDDM_ESC1CSErrCFS_flg) -> [VDDM_ESC1CSErrCFS_flg]
  TQD/34(VDDM_ESC1RCErrCFS_flg) -> [VDDM_ESC1RCErrCFS_flg]
  TQD/33(VDDM_ESC1NoComCFS_flg) -> [VDDM_ESC1NoComCFS_flg]
  TQD/32(VDDM_ESC7CSErrCFS_flg) -> [VDDM_ESC7CSErrCFS_flg]
  TQD/31(VDDM_ESC7RCErrCFS_flg) -> [VDDM_ESC7RCErrCFS_flg]
  TQD/30(VDDM_ESC7NoComCFS_flg) -> [VDDM_ESC7NoComCFS_flg]
  TQD/29(VDDM_MCUR1CSErrCFS_flg) -> [VDDM_MCUR1CSErrCFS_flg]
  TQD/28(VDDM_MCUR1RCErrCFS_flg) -> [VDDM_MCUR1RCErrCFS_flg]
  TQD/27(VDDM_MCUR1NoComCFS_flg) -> [VDDM_MCUR1NoComCFS_flg]
  TQD/26(VDDM_MCUF1CSErrCFS_flg) -> [VDDM_MCUF1CSErrCFS_flg]
  TQD/25(VDDM_MCUF1RCErrCFS_flg) -> [VDDM_MCUF1RCErrCFS_flg]
  TQD/24(VDDM_MCUF1NoComCFS_flg) -> [VDDM_MCUF1NoComCFS_flg]
  [VDDM_ESC5CSErr_flg] -> TQD/27(VDDM_ESC5CSErr_flg)
  TQD/20(VDDM_ESC5RCErrDTC_raw32) -> [VDDM_ESC5RCErrDTC_raw32]
  TQD/12(VDDM_MCUF1CSErrDTC_raw32) -> [VDDM_MCUF1CSErrDTC_raw32]
  TQD/1(VDDM_APS1SigOoRDTC_raw32) -> [VDDM_APS1SigOoRDTC_raw32]
  TQD/17(VDDM_ESC7CSErrDTC_raw32) -> [VDDM_ESC7CSErrDTC_raw32]
  [No_CAN1_BUS_OFF] -> TQD/9(No_CAN1_BUS_OFF)
  TQD/14(VDDM_Shifter1RCErrDTC_raw32) -> [VDDM_Shifter1RCErrDTC_raw32]
  [VINP_FrEDUDrtSta_flg] -> TQD/28(VINP_FrEDUDrtSta_flg)
  TQD/19(VDDM_ESC1CSErrDTC_raw32) -> [VDDM_ESC1CSErrDTC_raw32]
  TQD/18(VDDM_ESC1RCErrDTC_raw32) -> [VDDM_ESC1RCErrDTC_raw32]
  [VINP_RrEDUDrtSta_flg] -> TQD/32(VINP_RrEDUDrtSta_flg)
  [VDDM_MCUR1RCErr_flg] -> TQD/18(VDDM_MCUR1RCErr_flg)
  [VINP_CANMsgValidMCUF1_flg] -> TQD/10(VINP_CANMsgValidMCUF1_flg)
  TQD/10(VDDM_MCUF1RCErrDTC_raw32) -> [VDDM_MCUF1RCErrDTC_raw32]
  [VDDM_ESC1RCErr_flg] -> TQD/24(VDDM_ESC1RCErr_flg)
  TQD/13(VDDM_MCUR1CSErrDTC_raw32) -> [VDDM_MCUR1CSErrDTC_raw32]
  [VDDM_ESC1CSErr_flg] -> TQD/25(VDDM_ESC1CSErr_flg)
  [VINP_RrEDURealTMTq_Nm] -> TQD/33(VINP_RrEDURealTMTq_Nm)
  TQD/21(VDDM_ESC5CSErrDTC_raw32) -> [VDDM_ESC5CSErrDTC_raw32]
  TQD/22(VDDM_FrMCUTqErrDTC_raw32) -> [VDDM_FrMCUTqErrDTC_raw32]
  [task_time_s] -> TQD/6(task_time_s)
  [DTC_clear_request] -> TQD/7(DTC_clear_request)
  [VDDM_Shifter1CSErr_flg] -> TQD/21(VDDM_Shifter1CSErr_flg)
  TQD/15(VDDM_Shifter1CSErrDTC_raw32) -> [VDDM_Shifter1CSErrDTC_raw32]
  TQD/16(VDDM_ESC7RCErrDTC_raw32) -> [VDDM_ESC7RCErrDTC_raw32]
  [VINP_CANMsgValidShifter1_flg] -> TQD/12(VINP_CANMsgValidShifter1_flg)
  TQD/7(VDDM_ESC7NoComDTC_raw32) -> [VDDM_ESC7NoComDTC_raw32]
  [VDDM_ESC5RCErr_flg] -> TQD/26(VDDM_ESC5RCErr_flg)
  [VDDM_ESC7CSErr_flg] -> TQD/23(VDDM_ESC7CSErr_flg)
  [VTQR_RrTMTqReq_Nm] -> TQD/34(VTQR_RrTMTqReq_Nm)
  [VDHP_EAPS12RangeSta_enum] -> TQD/4(VDHP_EAPS12RangeSta_enum)
  [VDDM_MCUR1CSErr_flg] -> TQD/19(VDDM_MCUR1CSErr_flg)
  TQD/9(VDDM_ESC5NoComDTC_raw32) -> [VDDM_ESC5NoComDTC_raw32]
  [VDDM_Shifter1RCErr_flg] -> TQD/20(VDDM_Shifter1RCErr_flg)
  [VINP_CANMsgValidESC5_flg] -> TQD/15(VINP_CANMsgValidESC5_flg)
  TQD/3(VDDM_APSCorrErrDTC_raw32) -> [VDDM_APSCorrErrDTC_raw32]
  TQD/6(VDDM_Shifter1NoComDTC_raw32) -> [VDDM_Shifter1NoComDTC_raw32]
  TQD/4(VDDM_MCUF1NoComDTC_raw32) -> [VDDM_MCUF1NoComDTC_raw32]
  [VDDM_MCUF1RCErr_flg] -> TQD/16(VDDM_MCUF1RCErr_flg)
  [VINP_CANMsgValidMCUR1_flg] -> TQD/11(VINP_CANMsgValidMCUR1_flg)
  TQD/8(VDDM_ESC1NoComDTC_raw32) -> [VDDM_ESC1NoComDTC_raw32]
  [VDHP_EAPCRBAD_flg] -> TQD/5(VDHP_EAPCRBAD_flg)
  [VTQR_FrTMTqReq_Nm] -> TQD/31(VTQR_FrTMTqReq_Nm)
  [VINP_VehSpeed_kph] -> TQD/29(VINP_VehSpeed_kph)
  [VINP_CANMsgValidESC7_flg] -> TQD/13(VINP_CANMsgValidESC7_flg)
  TQD/11(VDDM_MCUR1RCErrDTC_raw32) -> [VDDM_MCUR1RCErrDTC_raw32]
  [No_CAN3_BUS_OFF] -> TQD/8(No_CAN3_BUS_OFF)
  [VINP_CANMsgValidESC1_flg] -> TQD/14(VINP_CANMsgValidESC1_flg)
  [VDDM_ESC7RCErr_flg] -> TQD/22(VDDM_ESC7RCErr_flg)
  [VDDM_MCUF1CSErr_flg] -> TQD/17(VDDM_MCUF1CSErr_flg)
  [VPMM_PwrStaSW_enum] -> TQD/1(VPMM_SysPwrSta_enum)
  TQD/2(VDDM_APS2SigOoRDTC_raw32) -> [VDDM_APS2SigOoRDTC_raw32]
  TQD/5(VDDM_MCUR1NoComDTC_raw32) -> [VDDM_MCUR1NoComDTC_raw32]
  TQD/23(VDDM_RrMCUTqErrDTC_raw32) -> [VDDM_RrMCUTqErrDTC_raw32]
  [VINP_FrEDURealTMTq_Nm] -> TQD/30(VINP_FrEDURealTMTq_Nm)
  [VINP_VehSpeed_kph] -> VMC_DDM/26(VINP_VehSpeed_kph)
  [VDDM_EDriveSysErrPMM_flg] -> Logical Operator5/2
  [VDDM_EDriveSysErrVMC_flg] -> Logical Operator5/1
  [VDDM_CCUSigErrDetDTC_raw32] -> VDDM_CCUSigErrDetDTC_raw32/1
  [VDDM_FCM5CSErrDTC_raw32] -> VDDM_FCM5CSErrDTC_raw32/1
  [VDDM_FCM5NoComDTC_raw32] -> VDDM_FCM5NoComDTC_raw32/1
  [VDDM_RrMCUSigErrDetDTC_raw32] -> VDDM_RrMCUSigErrDetDTC_raw32/1
  [VDDM_ACCAccelCmdErrDetDTC_raw32] -> VDDM_ACCAccelCmdErrDetDTC_raw32/1
  [VDDM_VCUACCErr_flg] -> VDDM_VCUACCErr_flg/1
  [VDDM_BMSSigErrDetDTC_raw32] -> VDDM_BMSSigErrDetDTC_raw32/1
  [VDDM_FCM4NoComDTC_raw32] -> VDDM_FCM4NoComDTC_raw32/1
  [VDDM_ACCMalfuncDetDTC_raw32] -> VDDM_ACCMalfuncDetDTC_raw32/1
  [VDDM_CCMalfuncDetDTC_raw32] -> VDDM_CCMalfuncDetDTC_raw32/1
  [VDDM_MSAMalfuncDetDTC_raw32] -> VDDM_MSAMalfuncDetDTC_raw32/1
  [VDDM_ZoneSCPNoComDTC_raw32] -> VDDM_ZoneSCPNoComDTC_raw32/1
  [VDDM_FrMCUSigErrDetDTC_raw32] -> VDDM_FrMCUSigErrDetDTC_raw32/1
  [VDDM_VCUISAErr_flg] -> VDDM_VCUISAErr_flg/1
  [VDDM_FCM4CSErrDTC_raw32] -> VDDM_FCM4CSErrDTC_raw32/1
  [VDDM_FCMACCSigErrDetDTC_raw32] -> VDDM_FCMACCSigErrDetDTC_raw32/1
  [VDDM_ISAMalfuncDetDTC_raw32] -> VDDM_ISAMalfuncDetDTC_raw32/1
  [VDDM_FCM3CSErrDTC_raw32] -> VDDM_FCM3CSErrDTC_raw32/1
  [VDDM_FCM3RCErrDTC_raw32] -> VDDM_FCM3RCErrDTC_raw32/1
  [VDDM_FCM3NoComDTC_raw32] -> VDDM_FCM3NoComDTC_raw32/1
  [VDDM_FCM2CSErrDTC_raw32] -> VDDM_FCM2CSErrDTC_raw32/1
  [VDDM_FCM2RCErrDTC_raw32] -> VDDM_FCM2RCErrDTC_raw32/1
  [VDDM_FCM2NoComDTC_raw32] -> VDDM_FCM2NoComDTC_raw32/1
  [VDDM_ESC5NoComCFS_flg] -> VMC_DDM/47(VDDM_ESC5NoComCFS_flg)
  [VDDM_ESC1NoComCFS_flg] -> VMC_DDM/44(VDDM_ESC1NoComCFS_flg)
  [VDDM_ESC7NoComCFS_flg] -> VMC_DDM/41(VDDM_ESC7NoComCFS_flg)
  [VDDM_MCUR1NoComCFS_flg] -> VMC_DDM/32(VDDM_MCUR1NoComCFS_flg)
  [VDDM_MCUF1NoComCFS_flg] -> VMC_DDM/27(VDDM_MCUF1NoComCFS_flg)
  [VDDM_C3CCU2CSCFS_flg] -> VMC_DDM/37(VDDM_C3CCU2CSCFS_flg)
  [VDDM_C3CCU2RCCFS_flg] -> VMC_DDM/36(VDDM_C3CCU2RCCFS_flg)
  [VDDM_C3CCU2LCCFS_flg] -> VMC_DDM/35(VDDM_C3CCU2LCCFS_flg)
  [VDDM_C3BMS6CSCFS_flg] -> VMC_DDM/19(VDDM_C3BMS6CSCFS_flg)
  [VDDM_C3BMS6RCCFS_flg] -> VMC_DDM/18(VDDM_C3BMS6RCCFS_flg)
  [VDDM_C3BMS6LCCFS_flg] -> VMC_DDM/17(VDDM_C3BMS6LCCFS_flg)
  VVMC_ADASActive_flg/1 -> VMC_DDM/39(VVMC_ADASActive_flg)
  VINP_ZoneSpdCtrlMode_enum/1 -> VMC_DDM/50(VINP_ZoneSpdCtrlMode_enum)
  VDDM_FCM5NoCom_flg/1 -> VMC_DDM/15(VDDM_FCM5NoCom_flg)
  VINP_ACCRequireAccel_mps2/1 -> VMC_DDM/40(VINP_ACCRequireAccel_mps2)
  VINP_VehSpeed_kph/1 -> [VINP_VehSpeed_kph]
  VINP_ADASACCSta_enum/1 -> VMC_DDM/7(VINP_ADASACCSta_enum)
  [VINP_DCDCFaultSta_enum] -> VMC_DDM/38(VINP_DCDCFaultSta_enum)
  [VINP_DCDCFaultSta_enum] -> PMM/18(VINP_DCDCFaultSta_enum)
  [VINP_MCUWarnR_enum] -> VMC_DDM/31(VINP_MCUWarnR_enum)
  [VINP_MCUWarnF_enum] -> VMC_DDM/30(VINP_MCUWarnF_enum)
  [VINP_MCUWarnR_enum] -> PMM/21(VINP_MCUWarnR_enum)
  [VINP_MCUWarnF_enum] -> PMM/20(VINP_MCUWarnF_enum)
  [VINP_BMSWarn8_flg] -> VMC_DDM/20(VINP_BMSWarn8_flg)
  [VINP_BMSWarn7_flg] -> VMC_DDM/21(VINP_BMSWarn7_flg)
  [VINP_BMSWarn6_flg] -> VMC_DDM/22(VINP_BMSWarn6_flg)
  [VINP_BMSWarn5_flg] -> VMC_DDM/23(VINP_BMSWarn5_flg)
  [VINP_BMSWarn4_flg] -> VMC_DDM/24(VINP_BMSWarn4_flg)
  [VINP_BMSWarn4_flg] -> PMM/13(VINP_BMSWarn4_flg)
  VINP_BMSWarn4_flg/1 -> [VINP_BMSWarn4_flg]
  [VINP_BMSWarn8_flg] -> PMM/17(VINP_BMSWarn8_flg)
  [VINP_BMSWarn7_flg] -> PMM/16(VINP_BMSWarn7_flg)
  [VINP_BMSWarn6_flg] -> PMM/15(VINP_BMSWarn6_flg)
  [VINP_BMSWarn5_flg] -> PMM/14(VINP_BMSWarn5_flg)
  VINP_BMSWarn8_flg/1 -> [VINP_BMSWarn8_flg]
  VINP_BMSWarn7_flg/1 -> [VINP_BMSWarn7_flg]
  VINP_BMSWarn6_flg/1 -> [VINP_BMSWarn6_flg]
  VINP_BMSWarn5_flg/1 -> [VINP_BMSWarn5_flg]
  VINP_CANMsgValidFCM4_flg/1 -> Logical Operator2/1
  VINP_CANMsgValidFCM3_flg/1 -> Logical Operator1/1
  VINP_CANMsgValidFCM2_flg/1 -> Logical Operator/1
  No_CAN_BUS_OFF/1 -> VMC_DDM/5(No_CAN_BUS_OFF)
  [No_CAN3_BUS_OFF] -> VMC_DDM/52(No_CAN3_BUS_OFF)
  [No_CAN1_BUS_OFF] -> VMC_DDM/51(No_CAN1_BUS_OFF)
  No_CAN4_BUS_OFF/1 -> VMC_DDM/53(No_CAN4_BUS_OFF)
  VDDM_ZoneSCPNoCom_flg/1 -> VMC_DDM/25(VDDM_ZoneSCPNoCom_flg)
  VDDM_FCM5CSErr_flg/1 -> VMC_DDM/16(VDDM_FCM5CSErr_flg)
  VDDM_FCM4CSErr_flg/1 -> VMC_DDM/14(VDDM_FCM4CSErr_flg)
  VDDM_FCM3CSErr_flg/1 -> VMC_DDM/11(VDDM_FCM3CSErr_flg)
  VDDM_FCM3RCErr_flg/1 -> VMC_DDM/10(VDDM_FCM3RCErr_flg)
  VDDM_FCM2CSErr_flg/1 -> VMC_DDM/4(VDDM_FCM2CSErr_flg)
  VDDM_FCM2RCErr_flg/1 -> VMC_DDM/3(VDDM_FCM2RCErr_flg)
  VINP_ADASISASta_enum/1 -> VMC_DDM/12(VINP_ADASISASta_enum)
  [VPMM_PowerSta_enum] -> VMC_DDM/6(VPMM_PowerSta_enum)
  [DTC_clear_request] -> VMC_DDM/8(DTC_clear_request)
  VMC_DDM/24(VDDM_EDriveSysErrVMC_flg) -> [VDDM_EDriveSysErrVMC_flg]
  VMC_DDM/23(VDDM_VCUISAErr_flg) -> [VDDM_VCUISAErr_flg]
  VMC_DDM/22(VDDM_VCUACCErr_flg) -> [VDDM_VCUACCErr_flg]
  VMC_DDM/21(VDDM_ISAMalfuncDetDTC_raw32) -> [VDDM_ISAMalfuncDetDTC_raw32]
  VMC_DDM/20(VDDM_MSAMalfuncDetDTC_raw32) -> [VDDM_MSAMalfuncDetDTC_raw32]
  VMC_DDM/19(VDDM_CCMalfuncDetDTC_raw32) -> [VDDM_CCMalfuncDetDTC_raw32]
  VMC_DDM/18(VDDM_ACCMalfuncDetDTC_raw32) -> [VDDM_ACCMalfuncDetDTC_raw32]
  VMC_DDM/17(VDDM_ACCAccelCmdErrDetDTC_raw32) -> [VDDM_ACCAccelCmdErrDetDTC_raw32]
  VMC_DDM/16(VDDM_CCUSigErrDetDTC_raw32) -> [VDDM_CCUSigErrDetDTC_raw32]
  VMC_DDM/15(VDDM_RrMCUSigErrDetDTC_raw32) -> [VDDM_RrMCUSigErrDetDTC_raw32]
  VMC_DDM/14(VDDM_FrMCUSigErrDetDTC_raw32) -> [VDDM_FrMCUSigErrDetDTC_raw32]
  VMC_DDM/13(VDDM_FCMACCSigErrDetDTC_raw32) -> [VDDM_FCMACCSigErrDetDTC_raw32]
  VMC_DDM/12(VDDM_BMSSigErrDetDTC_raw32) -> [VDDM_BMSSigErrDetDTC_raw32]
  VMC_DDM/11(VDDM_ZoneSCPNoComDTC_raw32) -> [VDDM_ZoneSCPNoComDTC_raw32]
  VMC_DDM/10(VDDM_FCM5CSErrDTC_raw32) -> [VDDM_FCM5CSErrDTC_raw32]
  VMC_DDM/9(VDDM_FCM5NoComDTC_raw32) -> [VDDM_FCM5NoComDTC_raw32]
  VMC_DDM/8(VDDM_FCM4CSErrDTC_raw32) -> [VDDM_FCM4CSErrDTC_raw32]
  VMC_DDM/7(VDDM_FCM4NoComDTC_raw32) -> [VDDM_FCM4NoComDTC_raw32]
  VMC_DDM/6(VDDM_FCM3CSErrDTC_raw32) -> [VDDM_FCM3CSErrDTC_raw32]
  VMC_DDM/5(VDDM_FCM3RCErrDTC_raw32) -> [VDDM_FCM3RCErrDTC_raw32]
  VMC_DDM/4(VDDM_FCM3NoComDTC_raw32) -> [VDDM_FCM3NoComDTC_raw32]
  VMC_DDM/3(VDDM_FCM2CSErrDTC_raw32) -> [VDDM_FCM2CSErrDTC_raw32]
  VMC_DDM/2(VDDM_FCM2RCErrDTC_raw32) -> [VDDM_FCM2RCErrDTC_raw32]
  VMC_DDM/1(VDDM_FCM2NoComDTC_raw32) -> [VDDM_FCM2NoComDTC_raw32]
  [task_time_s] -> VMC_DDM/1(task_time_s)
  [VDDM_FCLUSSDTC_raw32] -> VDDM_FCLUSSDTC_raw32/1
  [VDDM_RLLUSSDTC_raw32] -> VDDM_RLLUSSDTC_raw32/1
  [VDDM_RMLUSSDTC_raw32] -> VDDM_RMLUSSDTC_raw32/1
  [VDDM_FMLUSSDTC_raw32] -> VDDM_FMLUSSDTC_raw32/1
  [VDDM_RCLUSSDTC_raw32] -> VDDM_RCLUSSDTC_raw32/1
  [VDDM_RMRUSSDTC_raw32] -> VDDM_RMRUSSDTC_raw32/1
  [VDDM_RCRUSSDTC_raw32] -> VDDM_RCRUSSDTC_raw32/1
  [VDDM_FMRUSSDTC_raw32] -> VDDM_FMRUSSDTC_raw32/1
  [VDDM_RLRUSSDTC_raw32] -> VDDM_RLRUSSDTC_raw32/1
  [VDDM_FCRUSSDTC_raw32] -> VDDM_FCRUSSDTC_raw32/1
  [VDDM_FLRUSSDTC_raw32] -> VDDM_FLRUSSDTC_raw32/1
  [VDDM_FLLUSSDTC_raw32] -> VDDM_FLLUSSDTC_raw32/1
  [VPMM_PwrStaSW_enum] -> APM/14(VPMM_SysPwrSta_enum)
  VAPM_USSStaFLL_flg/1 -> APM/9(VAPM_USSStaFLL_flg)
  APM/1(VDDM_FCLUSSDTC_raw32) -> [VDDM_FCLUSSDTC_raw32]
  APM/11(VDDM_RLLUSSDTC_raw32) -> [VDDM_RLLUSSDTC_raw32]
  APM/5(VDDM_RCLUSSDTC_raw32) -> [VDDM_RCLUSSDTC_raw32]
  VAPM_USSStaRMR_flg/1 -> APM/7(VAPM_USSStaRMR_flg)
  APM/6(VDDM_RMLUSSDTC_raw32) -> [VDDM_RMLUSSDTC_raw32]
  VAPM_USSStaRLR_flg/1 -> APM/12(VAPM_USSStaRLR_flg)
  APM/4(VDDM_FCRUSSDTC_raw32) -> [VDDM_FCRUSSDTC_raw32]
  APM/9(VDDM_FLLUSSDTC_raw32) -> [VDDM_FLLUSSDTC_raw32]
  APM/7(VDDM_RMRUSSDTC_raw32) -> [VDDM_RMRUSSDTC_raw32]
  VAPM_USSStaFMR_flg/1 -> APM/3(VAPM_USSStaFMR_flg)
  VAPM_USSStaFLR_flg/1 -> APM/10(VAPM_USSStaFLR_flg)
  APM/8(VDDM_RCRUSSDTC_raw32) -> [VDDM_RCRUSSDTC_raw32]
  VAPM_USSStaRLL_flg/1 -> APM/11(VAPM_USSStaRLL_flg)
  VAPM_USSStaRCR_flg/1 -> APM/8(VAPM_USSStaRCR_flg)
  VAPM_USSStaRCL_flg/1 -> APM/5(VAPM_USSStaRCL_flg)
  APM/10(VDDM_FLRUSSDTC_raw32) -> [VDDM_FLRUSSDTC_raw32]
  VAPM_USSStaFCR_flg/1 -> APM/4(VAPM_USSStaFCR_flg)
  VAPM_USSStaRML_flg/1 -> APM/6(VAPM_USSStaRML_flg)
  APM/12(VDDM_RLRUSSDTC_raw32) -> [VDDM_RLRUSSDTC_raw32]
  VAPM_USSStaFCL_flg/1 -> APM/1(VAPM_USSStaFCL_flg)
  VAPM_USSStaFML_flg/1 -> APM/2(VAPM_USSStaFML_flg)
  APM/3(VDDM_FMRUSSDTC_raw32) -> [VDDM_FMRUSSDTC_raw32]
  APM/2(VDDM_FMLUSSDTC_raw32) -> [VDDM_FMLUSSDTC_raw32]
  [DTC_clear_request] -> APM/13(DTC_clear_request)
  Data Type Conversion56/1 -> [DTC_clear_request]
  [DTC_clear_request] -> BCM/6(DTC_clear_request)
  VPMM_PowerUpState_enum/1 -> PMM/73(VPMM_PowerUpState_enum)
  [VDDM_ESC1NoComDTC_raw32] -> Data Type Conversion55/1
  Data Type Conversion55/1 -> Chart/31(VDDM_ESC1NoComCFS_flg)
  Data Type Conversion54/1 -> Chart/34(VDDM_ESC5NoComCFS_flg)
  [VDDM_ESC5NoComDTC_raw32] -> Data Type Conversion54/1
  [VDDM_ESC7NoComDTC_raw32] -> Data Type Conversion53/1
  Data Type Conversion53/1 -> Chart/37(VDDM_ESC7NoComCFS_flg)
  Data Type Conversion52/1 -> Chart/57(VDDM_MCUF1NoComCFS_flg)
  [VDDM_MCUF1NoComDTC_raw32] -> Data Type Conversion52/1
  [VDDM_MCUR1NoComDTC_raw32] -> Data Type Conversion51/1
  Data Type Conversion51/1 -> Chart/60(VDDM_MCUR1NoComCFS_flg)
  Data Type Conversion50/1 -> Chart/68(VDDM_Shifter1NoComCFS_flg)
  [VDDM_Shifter1NoComDTC_raw32] -> Data Type Conversion50/1
  VINP_CANMsgValidMCUR1_flg/1 -> [VINP_CANMsgValidMCUR1_flg]
  VINP_CANMsgValidESC7_flg/1 -> [VINP_CANMsgValidESC7_flg]
  VINP_CANMsgValidMCUF1_flg/1 -> [VINP_CANMsgValidMCUF1_flg]
  VINP_AccelPedal1Vol_V/1 -> TQD/2(VINP_AccelPedal1Vol_V)
  VINP_CANMsgValidESC1_flg/1 -> [VINP_CANMsgValidESC1_flg]
  VINP_CANMsgValidESC5_flg/1 -> [VINP_CANMsgValidESC5_flg]
  [VDDM_Shifter1NoComDTC_raw32] -> VDDM_Shifter1NoComDTC_raw32/1
  VINP_CANMsgValidShifter1_flg/1 -> [VINP_CANMsgValidShifter1_flg]
  [VDDM_ESC7NoComDTC_raw32] -> VDDM_ESC7NoComDTC_raw32/1
  [VDDM_ESC5NoComDTC_raw32] -> VDDM_ESC5NoComDTC_raw32/1
  [VDDM_ESC1NoComDTC_raw32] -> VDDM_ESC1NoComDTC_raw32/1
  [VDDM_MCUR1NoComDTC_raw32] -> VDDM_MCUR1NoComDTC_raw32/1
  VINP_AccelPedal2Vol_V/1 -> TQD/3(VINP_AccelPedal2Vol_V)
  [VDDM_MCUF1NoComDTC_raw32] -> VDDM_MCUF1NoComDTC_raw32/1
  Constant1/1 -> Switch/3
  Chart/1(VDDM_VehMalfunLevel_enum) -> Switch/1
  Constant15/1 -> Switch/2
  [VDDM_DiagFLTSDTC_raw32] -> VDDM_DiagFLTSDTC_raw32/1
  [VDDM_DiagFRTSDTC_raw32] -> VDDM_DiagFRTSDTC_raw32/1
  [VDDM_DiagRLTSDTC_raw32] -> VDDM_DiagRLTSDTC_raw32/1
  [VDDM_DiagHCrashDTC_raw32] -> VDDM_DiagHCrashDTC_raw32/1
  [VDDM_DiagRRTSDTC_raw32] -> VDDM_DiagRRTSDTC_raw32/1
  BCM/5(VDDM_DiagRRTSDTC_raw32) -> [VDDM_DiagRRTSDTC_raw32]
  BCM/4(VDDM_DiagRLTSDTC_raw32) -> [VDDM_DiagRLTSDTC_raw32]
  BCM/3(VDDM_DiagFRTSDTC_raw32) -> [VDDM_DiagFRTSDTC_raw32]
  BCM/2(VDDM_DiagFLTSDTC_raw32) -> [VDDM_DiagFLTSDTC_raw32]
  VBCM_DiagRRTS_flg/1 -> BCM/5(VBCM_DiagRRTS_flg)
  VBCM_DiagRLTS_flg/1 -> BCM/4(VBCM_DiagRLTS_flg)
  VBCM_DiagFRTS_flg/1 -> BCM/3(VBCM_DiagFRTS_flg)
  VBCM_DiagFLTS_flg/1 -> BCM/2(VBCM_DiagFLTS_flg)
  BCM/1(VDDM_DiagHCrashDTC_raw32) -> [VDDM_DiagHCrashDTC_raw32]
  VBCM_DiagHCrash_flg/1 -> BCM/1(VBCM_DiagHCrash_flg)
  DTC_clear_request/1 -> Data Type Conversion56/1
  Data Type Conversion49/1 -> Equal/1
  [VPMM_PwrStaSW_enum] -> Data Type Conversion49/1
  Latch/1 -> Detect Increase/1
  Detect Increase/1 -> VDDM_EnterNewOperCyc_flg/1  "VDDM_EnterNewOperCyc_flg"
  Equal/1 -> Latch/1
  Constant/1 -> Equal/2
  [VDDM_APSCorrErrDTC_raw32] -> VDDM_APSCorrErrDTC_raw32/1
  [VDDM_APS2SigOoRDTC_raw32] -> VDDM_APS2SigOoRDTC_raw32/1
  [VDDM_APS1SigOoRDTC_raw32] -> VDDM_APS1SigOoRDTC_raw32/1
  [VDHP_EAPS12RangeSta_enum] -> PMM/63(VDHP_EAPS12RangeSta_enum)
  Data Type Conversion48/1 -> Chart/76(VDDM_APSCorrErrCFS_flg)
  [VDDM_APSCorrErrDTC_raw32] -> Data Type Conversion48/1
  Data Type Conversion45/1 -> Chart/75(VDDM_APS2SigOoRCFS_flg)
  [VDDM_APS2SigOoRDTC_raw32] -> Data Type Conversion45/1
  Data Type Conversion44/1 -> Chart/74(VDDM_APS1SigOoRCFS_flg)
  [VDDM_APS1SigOoRDTC_raw32] -> Data Type Conversion44/1
  VDHP_EAPS12RangeSta_enum/1 -> [VDHP_EAPS12RangeSta_enum]
  VDHP_EAPCRBAD_flg/1 -> [VDHP_EAPCRBAD_flg]
  Chart/3(VDDM_limphome_enum) -> Terminator1/1  "VDDM_limphome_enum"
  Chart/2(VDDM_EmergencyPwrDown_flg) -> Terminator/1  "VDDM_EmergencyPwrDown_flg"
  Switch/1 -> Terminator3/1
  [VDDM_ESC7CSErrCFS_flg] -> PMM/72(VDDM_ESC7CSErrCFS_flg)
  [VDDM_ESC7RCErrCFS_flg] -> PMM/71(VDDM_ESC7RCErrCFS_flg)
  [VDDM_ESC7NoComCFS_flg] -> PMM/70(VDDM_ESC7NoComCFS_flg)
  [VDDM_ESC5CSErrCFS_flg] -> PMM/69(VDDM_ESC5CSErrCFS_flg)
  [VDDM_ESC5RCErrCFS_flg] -> PMM/68(VDDM_ESC5RCErrCFS_flg)
  [VDDM_ESC5NoComCFS_flg] -> PMM/67(VDDM_ESC5NoComCFS_flg)
  [VDDM_MCUR1NoComCFS_flg] -> PMM/66(VDDM_MCUR1NoComCFS_flg)
  [VDDM_MCUF1NoComCFS_flg] -> PMM/65(VDDM_MCUF1NoComCFS_flg)
  Ground26/1 -> Chart/73(ZoneFrMalfunLevel_enum)
  [VINP_ZoneDrMalfunLevel_enum] -> Chart/72(ZoneDrMalfunLevel_enum)
  Data Type Conversion68/1 -> Chart/69(VDDM_Shifter1RCErrCFS_flg)
  Data Type Conversion67/1 -> Chart/67(VDDM_Shifter1CSErrCFS_flg)
  Data Type Conversion60/1 -> Chart/61(VDDM_MCUR1RCErrCFS_flg)
  Data Type Conversion59/1 -> Chart/59(VDDM_MCUR1CSErrCFS_flg)
  Data Type Conversion58/1 -> Chart/58(VDDM_MCUF1RCErrCFS_flg)
  Data Type Conversion57/1 -> Chart/56(VDDM_MCUF1CSErrCFS_flg)
  Data Type Conversion61/1 -> Chart/38(VDDM_ESC7RCErrCFS_flg)
  Data Type Conversion62/1 -> Chart/36(VDDM_ESC7CSErrCFS_flg)
  Data Type Conversion64/1 -> Chart/35(VDDM_ESC5RCErrCFS_flg)
  Data Type Conversion63/1 -> Chart/33(VDDM_ESC5CSErrCFS_flg)
  Data Type Conversion66/1 -> Chart/32(VDDM_ESC1RCErrCFS_flg)
  Data Type Conversion65/1 -> Chart/30(VDDM_ESC1CSErrCFS_flg)
  Data Type Conversion47/1 -> Chart/71(VDDM_TailgaSWCFS_flg)
  Data Type Conversion46/1 -> Chart/70(VDDM_HoodSWCFS_flg)
  Data Type Conversion43/1 -> Chart/66(VDDM_RRDoorSWCFS_flg)
  Data Type Conversion42/1 -> Chart/65(VDDM_RLDoorSWCFS_flg)
  Data Type Conversion41/1 -> Chart/64(VDDM_ONtoRdyCFS_flg)
  Data Type Conversion40/1 -> Chart/63(VDDM_OBC4PreCFS_flg)
  Data Type Conversion39/1 -> Chart/62(VDDM_MidLvSaChkCFS_flg)
  Data Type Conversion38/1 -> Chart/55(VDDM_MCUDisCFS_flg)
  Data Type Conversion37/1 -> Chart/54(VDDM_MCUActCFS_flg)
  Data Type Conversion36/1 -> Chart/53(VDDM_MCU4PreCFS_flg)
  Data Type Conversion35/1 -> Chart/1(VDDM_Lv4ErrCFS_flg)
  Data Type Conversion34/1 -> Chart/52(VDDM_Lv3ErrCFS_flg)
  Data Type Conversion33/1 -> Chart/51(VDDM_Lv2ErrCFS_flg)
  Data Type Conversion32/1 -> Chart/50(VDDM_Lv1ErrCFS_flg)
  Data Type Conversion23/1 -> Chart/49(VDDM_LVSupLoCFS_flg)
  Ground4/1 -> Chart/47(VDDM_LVChFrqCFS_flg)
  Data Type Conversion22/1 -> Chart/48(VDDM_LVSupHiCFS_flg)
  Data Type Conversion21/1 -> Chart/46(VDDM_KeyAuthCFS_flg)
  Data Type Conversion20/1 -> Chart/45(VDDM_IniLVLoCFS_flg)
  Data Type Conversion19/1 -> Chart/44(VDDM_HiLvSaChkCFS_flg)
  Data Type Conversion18/1 -> Chart/43(VDDM_HVRlyOpCFS_flg)
  Data Type Conversion31/1 -> Chart/42(VDDM_HVRlyCloCFS_flg)
  Data Type Conversion30/1 -> Chart/41(VDDM_HVB4PreCFS_flg)
  Data Type Conversion29/1 -> Chart/40(VDDM_FRDoorSWCFS_flg)
  Data Type Conversion28/1 -> Chart/39(VDDM_FLDoorSWCFS_flg)
  Data Type Conversion27/1 -> Chart/27(VDDM_DrStSWCFS_flg)
  Data Type Conversion26/1 -> Chart/26(VDDM_DCDCEnaCFS_flg)
  Data Type Conversion25/1 -> Chart/25(VDDM_DCDCDisCFS_flg)
  Data Type Conversion24/1 -> Chart/24(VDDM_DCDC4PreCFS_flg)
  Data Type Conversion17/1 -> Chart/23(VDDM_C3CCU2RCCFS_flg)
  Data Type Conversion16/1 -> Chart/22(VDDM_C3CCU2LCCFS_flg)
  Data Type Conversion15/1 -> Chart/21(VDDM_C3CCU2CSCFS_flg)
  Data Type Conversion14/1 -> Chart/20(VDDM_C3CCU1RCCFS_flg)
  Data Type Conversion13/1 -> Chart/19(VDDM_C3CCU1LCCFS_flg)
  Data Type Conversion12/1 -> Chart/18(VDDM_C3CCU1CSCFS_flg)
  Data Type Conversion11/1 -> Chart/17(VDDM_C3BMS6RCCFS_flg)
  Data Type Conversion10/1 -> Chart/16(VDDM_C3BMS6LCCFS_flg)
  Data Type Conversion9/1 -> Chart/15(VDDM_C3BMS6CSCFS_flg)
  Data Type Conversion8/1 -> Chart/14(VDDM_C3BMS1RCCFS_flg)
  Data Type Conversion7/1 -> Chart/13(VDDM_C3BMS1LCCFS_flg)
  Data Type Conversion6/1 -> Chart/12(VDDM_C3BMS1CSCFS_flg)
  Data Type Conversion5/1 -> Chart/11(VDDM_C1ABM1RCCFS_flg)
  Data Type Conversion4/1 -> Chart/10(VDDM_C1ABM1LCCFS_flg)
  Data Type Conversion3/1 -> Chart/9(VDDM_C1ABM1CSCFS_flg)
  Data Type Conversion2/1 -> Chart/8(VDDM_BrkSWNoBacCFS_flg)
  Data Type Conversion1/1 -> Chart/7(VDDM_BrkSWErrCFS_flg)
  Data Type Conversion/1 -> Chart/6(VDDM_BMSRdyCFS_flg)
  Ground3/1 -> Chart/5(VDDM_5vAPS2PwrErrCFS_flg)
  Ground1/1 -> Chart/3(VDDM_5vAPS1PwrErrCFS_flg)
  [VDDM_MidLvSaChkDTC_raw32] -> Data Type Conversion39/1
  [VDDM_OBC4PreDTC_raw32] -> Data Type Conversion40/1
  [VDDM_RLDoorSWDTC_raw32] -> Data Type Conversion42/1
  [VDDM_ONtoRdyDTC_raw32] -> Data Type Conversion41/1
  [VDDM_HoodSWDTC_raw32] -> Data Type Conversion46/1
  [VDDM_RRDoorSWDTC_raw32] -> Data Type Conversion43/1
  [VDDM_TailgaSWDTC_raw32] -> Data Type Conversion47/1
  [VDDM_MCUDisDTC_raw32] -> Data Type Conversion38/1
  [VDDM_Lv3ErrDTC_raw32] -> Data Type Conversion34/1
  [VDDM_Lv4ErrDTC_raw32] -> Data Type Conversion35/1
  [VDDM_MCUActDTC_raw32] -> Data Type Conversion37/1
  [VDDM_MCU4PreDTC_raw32] -> Data Type Conversion36/1
  [VDDM_Lv1ErrDTC_raw32] -> Data Type Conversion32/1
  [VDDM_Lv2ErrDTC_raw32] -> Data Type Conversion33/1
  [VDDM_C3CCU2LCDTC_raw32] -> Data Type Conversion16/1
  [VDDM_C3CCU2RCDTC_raw32] -> Data Type Conversion17/1
  [VDDM_DCDCDisDTC_raw32] -> Data Type Conversion25/1
  [VDDM_DCDC4PreDTC_raw32] -> Data Type Conversion24/1
  [VDDM_FLDoorSWDTC_raw32] -> Data Type Conversion28/1
  [VDDM_FRDoorSWDTC_raw32] -> Data Type Conversion29/1
  [VDDM_DrStSWDTC_raw32] -> Data Type Conversion27/1
  [VDDM_DCDCEnaDTC_raw32] -> Data Type Conversion26/1
  [VDDM_IniLVLoDTC_raw32] -> Data Type Conversion20/1
  [VDDM_KeyAuthDTC_raw32] -> Data Type Conversion21/1
  [VDDM_LVSupLoDTC_raw32] -> Data Type Conversion23/1
  [VDDM_LVSupHiDTC_raw32] -> Data Type Conversion22/1
  [VDDM_HVRlyOpDTC_raw32] -> Data Type Conversion18/1
  [VDDM_HiLvSaChkDTC_raw32] -> Data Type Conversion19/1
  [VDDM_HVRlyCloDTC_raw32] -> Data Type Conversion31/1
  [VDDM_HVB4PreDTC_raw32] -> Data Type Conversion30/1
  [VDDM_C3BMS1RCDTC_raw32] -> Data Type Conversion8/1
  [VDDM_C3BMS6CSDTC_raw32] -> Data Type Conversion9/1
  [VDDM_C3BMS6RCDTC_raw32] -> Data Type Conversion11/1
  [VDDM_C3BMS6LCDTC_raw32] -> Data Type Conversion10/1
  [VDDM_C3CCU1RCDTC_raw32] -> Data Type Conversion14/1
  [VDDM_C3CCU2CSDTC_raw32] -> Data Type Conversion15/1
  [VDDM_C3CCU1LCDTC_raw32] -> Data Type Conversion13/1
  [VDDM_C3CCU1CSDTC_raw32] -> Data Type Conversion12/1
  [VDDM_C1ABM1LCDTC_raw32] -> Data Type Conversion4/1
  [VDDM_C1ABM1RCDTC_raw32] -> Data Type Conversion5/1
  [VDDM_C3BMS1LCDTC_raw32] -> Data Type Conversion7/1
  [VDDM_C3BMS1CSDTC_raw32] -> Data Type Conversion6/1
  [VDDM_BrkSWNoBacDTC_raw32] -> Data Type Conversion2/1
  [VDDM_C1ABM1CSDTC_raw32] -> Data Type Conversion3/1
  [VDDM_BrkSWErrDTC_raw32] -> Data Type Conversion1/1
  [VDDM_TailgaSWDTC_raw32] -> VDDM_TailgaSWDTC_raw32/1
  [VDDM_HoodSWDTC_raw32] -> VDDM_HoodSWDTC_raw32/1
  [VDDM_RRDoorSWDTC_raw32] -> VDDM_RRDoorSWDTC_raw32/1
  [VDDM_FRDoorSWDTC_raw32] -> VDDM_FRDoorSWDTC_raw32/1
  [VDDM_RLDoorSWDTC_raw32] -> VDDM_RLDoorSWDTC_raw32/1
  [VDDM_FLDoorSWDTC_raw32] -> VDDM_FLDoorSWDTC_raw32/1
  [VDDM_DrStSWDTC_raw32] -> VDDM_DrStSWDTC_raw32/1
  [VDDM_LVSupHiDTC_raw32] -> VDDM_LVSupHiDTC_raw32/1
  [VDDM_LVSupLoDTC_raw32] -> VDDM_LVSupLoDTC_raw32/1
  [VDDM_IniLVLoDTC_raw32] -> VDDM_IniLVLoDTC_raw32/1
  [VDDM_OBC4PreDTC_raw32] -> VDDM_OBC4PreDTC_raw32/1
  [VDDM_MCUActDTC_raw32] -> VDDM_MCUActDTC_raw32/1
  [VDDM_HVRlyOpDTC_raw32] -> VDDM_HVRlyOpDTC_raw32/1
  [VDDM_DCDCDisDTC_raw32] -> VDDM_DCDCDisDTC_raw32/1
  [VDDM_MCUDisDTC_raw32] -> VDDM_MCUDisDTC_raw32/1
  [VDDM_MidLvSaChkDTC_raw32] -> VDDM_MidLvSaChkDTC_raw32/1
  [VDDM_HiLvSaChkDTC_raw32] -> VDDM_HiLvSaChkDTC_raw32/1
  [VDDM_DCDCEnaDTC_raw32] -> VDDM_DCDCEnaDTC_raw32/1
  [VDDM_BMSRdyDTC_raw32] -> VDDM_BMSRdyDTC_raw32/1
  [VDDM_HVRlyCloDTC_raw32] -> VDDM_HVRlyCloDTC_raw32/1
  [VDDM_DCDC4PreDTC_raw32] -> VDDM_DCDC4PreDTC_raw32/1
  [VDDM_MCU4PreDTC_raw32] -> VDDM_MCU4PreDTC_raw32/1
  [VDDM_HVB4PreDTC_raw32] -> VDDM_HVB4PreDTC_raw32/1
  [VDDM_ONtoRdyDTC_raw32] -> VDDM_ONtoRdyDTC_raw32/1
  [VDDM_KeyAuthDTC_raw32] -> VDDM_KeyAuthDTC_raw32/1
  [VDDM_BrkSWNoBacDTC_raw32] -> VDDM_BrkSWNoBacDTC_raw32/1
  [VDDM_BrkSWErrDTC_raw32] -> VDDM_BrkSWErrDTC_raw32/1
  [VDDM_Lv4ErrDTC_raw32] -> VDDM_Lv4ErrDTC_raw32/1
  [VDDM_Lv3ErrDTC_raw32] -> VDDM_Lv3ErrDTC_raw32/1
  [VDDM_Lv2ErrDTC_raw32] -> VDDM_Lv2ErrDTC_raw32/1
  [VDDM_Lv1ErrDTC_raw32] -> VDDM_Lv1ErrDTC_raw32/1
  [VDDM_C1ABM1LCDTC_raw32] -> VDDM_C1ABM1LCDTC_raw32/1
  [VDDM_C1ABM1CSDTC_raw32] -> VDDM_C1ABM1CSDTC_raw32/1
  [VDDM_C1ABM1RCDTC_raw32] -> VDDM_C1ABM1RCDTC_raw32/1
  [VDDM_C3CCU2LCDTC_raw32] -> VDDM_C3CCU2LCDTC_raw32/1
  [VDDM_C3CCU2CSDTC_raw32] -> VDDM_C3CCU2CSDTC_raw32/1
  [VDDM_C3CCU2RCDTC_raw32] -> VDDM_C3CCU2RCDTC_raw32/1
  [VDDM_C3CCU1LCDTC_raw32] -> VDDM_C3CCU1LCDTC_raw32/1
  [VDDM_C3CCU1CSDTC_raw32] -> VDDM_C3CCU1CSDTC_raw32/1
  [VDDM_C3CCU1RCDTC_raw32] -> VDDM_C3CCU1RCDTC_raw32/1
  [VDDM_C3BMS1LCDTC_raw32] -> VDDM_C3BMS1LCDTC_raw32/1
  [VDDM_C3BMS1CSDTC_raw32] -> VDDM_C3BMS1CSDTC_raw32/1
  [VDDM_C3BMS1RCDTC_raw32] -> VDDM_C3BMS1RCDTC_raw32/1
  [VDDM_C3BMS6LCDTC_raw32] -> VDDM_C3BMS6LCDTC_raw32/1
  [VDDM_C3BMS6CSDTC_raw32] -> VDDM_C3BMS6CSDTC_raw32/1
  [VDDM_C3BMS6RCDTC_raw32] -> VDDM_C3BMS6RCDTC_raw32/1
  PMM/46(VDDM_TailgaSWDTC_raw32) -> [VDDM_TailgaSWDTC_raw32]
  PMM/45(VDDM_HoodSWDTC_raw32) -> [VDDM_HoodSWDTC_raw32]
  PMM/44(VDDM_RRDoorSWDTC_raw32) -> [VDDM_RRDoorSWDTC_raw32]
  PMM/43(VDDM_FRDoorSWDTC_raw32) -> [VDDM_FRDoorSWDTC_raw32]
  PMM/42(VDDM_RLDoorSWDTC_raw32) -> [VDDM_RLDoorSWDTC_raw32]
  PMM/41(VDDM_FLDoorSWDTC_raw32) -> [VDDM_FLDoorSWDTC_raw32]
  PMM/40(VDDM_DrStSWDTC_raw32) -> [VDDM_DrStSWDTC_raw32]
  PMM/39(VDDM_LVSupHiDTC_raw32) -> [VDDM_LVSupHiDTC_raw32]
  PMM/38(VDDM_LVSupLoDTC_raw32) -> [VDDM_LVSupLoDTC_raw32]
  PMM/37(VDDM_IniLVLoDTC_raw32) -> [VDDM_IniLVLoDTC_raw32]
  PMM/36(VDDM_OBC4PreDTC_raw32) -> [VDDM_OBC4PreDTC_raw32]
  PMM/35(VDDM_MCUActDTC_raw32) -> [VDDM_MCUActDTC_raw32]
  PMM/34(VDDM_HVRlyOpDTC_raw32) -> [VDDM_HVRlyOpDTC_raw32]
  PMM/33(VDDM_DCDCDisDTC_raw32) -> [VDDM_DCDCDisDTC_raw32]
  PMM/32(VDDM_MCUDisDTC_raw32) -> [VDDM_MCUDisDTC_raw32]
  PMM/31(VDDM_MidLvSaChkDTC_raw32) -> [VDDM_MidLvSaChkDTC_raw32]
  PMM/30(VDDM_HiLvSaChkDTC_raw32) -> [VDDM_HiLvSaChkDTC_raw32]
  PMM/29(VDDM_DCDCEnaDTC_raw32) -> [VDDM_DCDCEnaDTC_raw32]
  PMM/28(VDDM_BMSRdyDTC_raw32) -> [VDDM_BMSRdyDTC_raw32]
  PMM/27(VDDM_HVRlyCloDTC_raw32) -> [VDDM_HVRlyCloDTC_raw32]
  PMM/26(VDDM_DCDC4PreDTC_raw32) -> [VDDM_DCDC4PreDTC_raw32]
  PMM/25(VDDM_MCU4PreDTC_raw32) -> [VDDM_MCU4PreDTC_raw32]
  PMM/24(VDDM_HVB4PreDTC_raw32) -> [VDDM_HVB4PreDTC_raw32]
  PMM/23(VDDM_ONtoRdyDTC_raw32) -> [VDDM_ONtoRdyDTC_raw32]
  PMM/22(VDDM_KeyAuthDTC_raw32) -> [VDDM_KeyAuthDTC_raw32]
  PMM/21(VDDM_BrkSWNoBacDTC_raw32) -> [VDDM_BrkSWNoBacDTC_raw32]
  PMM/20(VDDM_BrkSWErrDTC_raw32) -> [VDDM_BrkSWErrDTC_raw32]
  PMM/19(VDDM_Lv4ErrDTC_raw32) -> [VDDM_Lv4ErrDTC_raw32]
  PMM/18(VDDM_Lv3ErrDTC_raw32) -> [VDDM_Lv3ErrDTC_raw32]
  PMM/17(VDDM_Lv2ErrDTC_raw32) -> [VDDM_Lv2ErrDTC_raw32]
  PMM/16(VDDM_Lv1ErrDTC_raw32) -> [VDDM_Lv1ErrDTC_raw32]
  PMM/15(VDDM_C1ABM1LCDTC_raw32) -> [VDDM_C1ABM1LCDTC_raw32]
  PMM/14(VDDM_C1ABM1CSDTC_raw32) -> [VDDM_C1ABM1CSDTC_raw32]
  PMM/13(VDDM_C1ABM1RCDTC_raw32) -> [VDDM_C1ABM1RCDTC_raw32]
  PMM/12(VDDM_C3CCU2LCDTC_raw32) -> [VDDM_C3CCU2LCDTC_raw32]
  PMM/11(VDDM_C3CCU2CSDTC_raw32) -> [VDDM_C3CCU2CSDTC_raw32]
  PMM/10(VDDM_C3CCU2RCDTC_raw32) -> [VDDM_C3CCU2RCDTC_raw32]
  PMM/9(VDDM_C3CCU1LCDTC_raw32) -> [VDDM_C3CCU1LCDTC_raw32]
  PMM/8(VDDM_C3CCU1CSDTC_raw32) -> [VDDM_C3CCU1CSDTC_raw32]
  PMM/7(VDDM_C3CCU1RCDTC_raw32) -> [VDDM_C3CCU1RCDTC_raw32]
  PMM/6(VDDM_C3BMS1LCDTC_raw32) -> [VDDM_C3BMS1LCDTC_raw32]
  PMM/5(VDDM_C3BMS1CSDTC_raw32) -> [VDDM_C3BMS1CSDTC_raw32]
  PMM/4(VDDM_C3BMS1RCDTC_raw32) -> [VDDM_C3BMS1RCDTC_raw32]
  PMM/3(VDDM_C3BMS6LCDTC_raw32) -> [VDDM_C3BMS6LCDTC_raw32]
  PMM/2(VDDM_C3BMS6CSDTC_raw32) -> [VDDM_C3BMS6CSDTC_raw32]
  PMM/1(VDDM_C3BMS6RCDTC_raw32) -> [VDDM_C3BMS6RCDTC_raw32]
  [VDDM_BMSRdyDTC_raw32] -> Data Type Conversion/1
  [No_CAN1_BUS_OFF] -> PMM/61(No_CAN1_BUS_OFF)
  [No_CAN3_BUS_OFF] -> PMM/62(No_CAN3_BUS_OFF)
  [DTC_clear_request] -> PMM/64(DTC_clear_request)
  [VPMM_PwrStaSW_enum] -> PMM/31(VPMM_PwrStaSW_enum)
  [VPMM_PowerSta_enum] -> PMM/30(VPMM_PowerSta_enum)
  [task_time_s] -> PMM/1(task_time_s)
  No_CAN3_BUS_OFF/1 -> [No_CAN3_BUS_OFF]
  No_CAN1_BUS_OFF/1 -> [No_CAN1_BUS_OFF]
  VPMM_PwrStaSW_enum/1 -> [VPMM_PwrStaSW_enum]
  VPMM_PowerSta_enum/1 -> [VPMM_PowerSta_enum]
  task_time_s/1 -> [task_time_s]
  PMM/47(VDDM_EDriveSysErrPMM_flg) -> [VDDM_EDriveSysErrPMM_flg]
  VINP_AllowMovThd_OTA_enum/1 -> PMM/60(VINP_AllowMovThd_OTA_enum)
  VDKC_DKCAuthSta_enum/1 -> PMM/59(VDKC_DKCAuthSta_enum)
  VINP_TailgaSW/1 -> PMM/58(VINP_TailgaSW)
  VINP_HoodSW/1 -> PMM/57(VINP_HoodSW)
  VINP_RRAJARSW/1 -> PMM/56(VINP_RRAJARSW)
  VINP_RLAJARSW/1 -> PMM/55(VINP_RLAJARSW)
  VINP_FRAJARSW/1 -> PMM/54(VINP_FRAJARSW)
  VINP_FLAJARSW/1 -> PMM/53(VINP_FLAJARSW)
  VINP_DrStSW/1 -> PMM/52(VINP_DrStSW)
  VINP_BrakeLampSW_flg/1 -> PMM/51(VINP_BrakeLampSW_flg)
  VINP_BrakeSWGPIO_flg/1 -> PMM/50(VINP_BrakeSWGPIO_flg)
  VDDM_C1ABM1CSChk_flg/1 -> PMM/49(VDDM_C1ABM1CSChk_flg)
  VDDM_C1ABM1RCChk_flg/1 -> PMM/48(VDDM_C1ABM1RCChk_flg)
  VDDM_C3CCU2CSChk_flg/1 -> PMM/47(VDDM_C3CCU2CSChk_flg)
  VDDM_C3CCU2RCChk_flg/1 -> PMM/46(VDDM_C3CCU2RCChk_flg)
  VDDM_C3CCU1CSChk_flg/1 -> PMM/45(VDDM_C3CCU1CSChk_flg)
  VDDM_C3CCU1RCChk_flg/1 -> PMM/44(VDDM_C3CCU1RCChk_flg)
  VDDM_C3BMS1CSChk_flg/1 -> PMM/43(VDDM_C3BMS1CSChk_flg)
  VDDM_C3BMS1RCChk_flg/1 -> PMM/42(VDDM_C3BMS1RCChk_flg)
  VDDM_C3BMS6CSChk_flg/1 -> PMM/41(VDDM_C3BMS6CSChk_flg)
  VDDM_C3BMS6RCChk_flg/1 -> PMM/40(VDDM_C3BMS6RCChk_flg)
  VPMM_MCUReady4Pre_flg/1 -> PMM/39(VPMM_MCUReady4Pre_flg)
  VPMM_MCUReady_flg/1 -> PMM/38(VPMM_MCUReady_flg)
  VPMM_HVChrgPreActionErrSta_enum/1 -> PMM/37(VPMM_HVChrgPreActionErrSta_enum)
  VPMM_SafetyChkMLv_flg/1 -> PMM/36(VPMM_SafetyChkMLv_flg)
  VPMM_SafetyChkHLv_flg/1 -> PMM/35(VPMM_SafetyChkHLv_flg)
  VPMM_DrivetrainSelect_enum/1 -> [VPMM_DrivetrainSelect_enum]
  VPMM_PowerDownFault_enum/1 -> PMM/33(VPMM_PowerDownFault_enum)
  VPMM_PowerUpFault_enum/1 -> PMM/32(VPMM_PowerUpFault_enum)
  VINP_DrStdAErrSta_enum/1 -> PMM/29(VINP_DrStdAErrSta_enum)
  VINP_CANMsgValidBMS2_flg/1 -> PMM/28(VINP_CANMsgValidBMS2_flg)
  VINP_DCDCEnabled_flg/1 -> PMM/27(VINP_DCDCEnabled_flg)
  VINP_DCDCReady4Pre_flg/1 -> PMM/26(VINP_DCDCReady4Pre_flg)
  VINP_HVBContactorSta_flg/1 -> PMM/25(VINP_HVBContactorSta_flg)
  VINP_HVBattReady4Pre_enum/1 -> PMM/24(VINP_HVBattReady4Pre_enum)
  VINP_BMSREADY_flg/1 -> PMM/23(VINP_BMSREADY_flg)
  VINP_LVBattDet12V_V/1 -> [VINP_LVBattDet12V_V]
  VINP_MCUWarnR_enum/1 -> [VINP_MCUWarnR_enum]
  VINP_MCUWarnF_enum/1 -> [VINP_MCUWarnF_enum]
  VINP_OBCFaultSta_enum/1 -> PMM/19(VINP_OBCFaultSta_enum)
  VINP_DCDCFaultSta_enum/1 -> [VINP_DCDCFaultSta_enum]
  VINP_BMSWarn3_flg/1 -> PMM/12(VINP_BMSWarn3_flg)
  VINP_BMSWarn2_flg/1 -> PMM/11(VINP_BMSWarn2_flg)
  VINP_BMSWarn1_flg/1 -> PMM/10(VINP_BMSWarn1_flg)
  VINP_CANMsgValidCCU2_flg/1 -> PMM/9(VINP_CANMsgValidCCU2_flg)
  VINP_CANMsgValidCCU1_flg/1 -> PMM/8(VINP_CANMsgValidCCU1_flg)
  VINP_CANMsgValidBMS6_flg/1 -> PMM/7(VINP_CANMsgValidBMS6_flg)
  VINP_CANMsgValidBMS1_flg/1 -> PMM/6(VINP_CANMsgValidBMS1_flg)
  VINP_BrkSWSta_flg/1 -> PMM/5(VINP_BrkSWSta_flg)
  VINP_BrkPedalPos_pct/1 -> PMM/4(VINP_BrkPedalPos_pct)
  VINP_BrkPedalPosSta_enum/1 -> PMM/3(VINP_BrkPedalPosSta_enum)
  VINP_CANMsgValidABM1_flg/1 -> PMM/2(VINP_CANMsgValidABM1_flg)
  TQD/43(EDriveSysErr_VCUErr) -> [EDriveSysErr_VCUErr]
  TQD/44(EDriveSysErr_ShifterErr) -> [EDriveSysErr_ShifterErr]
  TQD/45(EngageP_Fail) -> [EngageP_Fail]
  [VINP_LVBattDet12V_V] -> PMM/22(VINP_LVBattDet12V_V)
  [VDDM_SysAllowReadySta_flg] -> VDDM_SysAllowReadySta_flg/1
  [VPMM_DrivetrainSelect_enum] -> PMM/34(VPMM_DrivetrainSelect_enum)
  [VPMM_DrivetrainSelect_enum] -> TQD/50(VPMM_DrivetrainSelect_enum)
  [VINP_BMSWarn4_flg] -> TQD/44(VINP_BMSWarn4_flg)
  [VINP_BMSWarn5_flg] -> TQD/45(VINP_BMSWarn5_flg)
  [VINP_BMSWarn6_flg] -> TQD/46(VINP_BMSWarn6_flg)
  [VINP_BMSWarn7_flg] -> TQD/47(VINP_BMSWarn7_flg)
  [VINP_BMSWarn8_flg] -> TQD/48(VINP_BMSWarn8_flg)
  [VINP_DCDCFaultSta_enum] -> TQD/49(VINP_DCDCFaultSta_enum)
  TQD/46(VDDM_LimpHomeActTmp_flg) -> [VDDM_LimpHomeActTmp_flg]
  [VDDM_LimpHomeActTmp_flg] -> VDDM_LimpHomeActTmp_flg/1
  Logical Operator5/1 -> Terminator2/1
  TQD/47(VDDM_EDriveSysErr_VCUErrTmp_flg) -> [VDDM_EDriveSysErr_VCUErrTmp_flg]
  [VDDM_EDriveSysErr_VCUErrTmp_flg] -> VDDM_EDriveSysErr_VCUErrTmp_flg/1
  VINP_CANMsgValidDKC1_flg/1 -> PMM/76(VINP_CANMsgValidDKC1_flg)
  VINP_CANMsgValidDKC2_flg/1 -> PMM/77(VINP_CANMsgValidDKC2_flg)
  TQD/48(VDDM_VehMalfunLevelTmp_enum) -> [VDDM_VehMalfunLevelTmp_enum]
  [VDDM_VehMalfunLevelTmp_enum] -> Data Type Conversion73/1
  Data Type Conversion73/1 -> VDDM_VehMalfunLevel_enum/1  "VDDM_VehMalfunLevel_enum"
